simulink library "ammclib_bam_S32K3xx"  (R2016a)
settings: Solver=VariableStepAuto  SolverMode=SingleTasking  StartTime=0.0  StopTime=10.0  RelTol=1e-3
undefined symbols (not defined in the file or in its folder): a1, a2, ADCMaxError, autoCalcEn, b0, b1, b2, cfg, dgain, escale, f16A1, f16A2, f16ADCMaxError, f16B0, f16B1, f16B2, f16C1, f16CC1sc, f16CC1sc_D, f16CC1sc_Q, f16CC2sc, f16CC2sc_D, f16CC2sc_Q, f16DerivGain, f16EGain, f16FiltCoef, f16HystOff, f16HystOn, f16IGain, f16IntegGain, f16IntegGain_D, f16IntegGain_Q, f16IntegGainQ, f16Kd, f16KLs, f16Kq, f16KRs, f16Limit, f16LowerLimit, f16LowerLimit_D, f16LowerLimit_Q, f16LowerLimitQ, f16ModIndex, f16OutValOff, f16OutValOn, f16PropGain, f16PropGain_D, f16PropGain_Q, f16PropGainQ, f16RampDown, f16RampUp, f16UGain, f16UpperLimit, f16UpperLimit_D, f16UpperLimit_Q, f16UpperLimitQ, f16WIGain, f32A1, f32A2, f32ADCMaxError ... (+180)
(part 2 of 50)

== system ammclib_bam_S32K3xx/AMCLIB/F16 ==
  AMCLIB_BemfObsrvDQ_F16 : Subsystem  StartFcn=|  TreatAsAtomicUnit=on  mask(AMCLIB_BemfObsrvDQ_F16){showStates=Hide (faster execution), resetStatesEnable=Pre-set according to the first set of inputs after reset, SampleTime=-1, intmethod=Trapezoidal, if0=350, iksi=1, Ld=3e-4, Lq=3e-4, Rs=0.33, mechspeed=3000, polepairs=1, uscale=15, escale=15, iscale=10, autoCalcEn=on, f16IGain=0, f16UGain=0, f16WIGain=0, f16EGain=0, s16Shift=0, f16CC1sc_D=0, f16CC2sc_D=0, f16UpperLimit_D=0, f16LowerLimit_D=0, f16CC1sc_Q=0, f16CC2sc_Q=0, f16UpperLimit_Q=0, f16LowerLimit_Q=0, u16NShift=0, SampleTime_1=NaN}
      | ts=get_param(gcb,'CompiledSampleTime');
      | if iscell(ts)
      |   ts=ts{1};
      |   if iscell(ts)
      |     ts=ts{1};
      |   end
      | end
      | ts=ts(1);
      | set_param(gcb,'SampleTime_1',num2str(ts));
      | p=Simulink.Mask.get(gcb);
      | hintText=p.getDialogControl('timeHint');
      | SampleTime=Simulink.data.evalinGlobal(bdroot,get_param(gcb,'SampleTime'));
      | p=Simulink.Mask.get(gcb);
      | autoCalcEn=get_param(gcb,'autoCalcEn');
      | if strcmp(autoCalcEn,'on')
      |   if SampleTime==-1
      |     hintText.Prompt='Caution: Implementation parameters depend on inherited sample time. Make sure that the sample time of the block''s inputs corresponds to the sampling period in the target application.';
      |   else
      |     hintText.Prompt='Caution: Implementation parameters depend on the sample time. Make sure that the simulation time step corresponds to the sampling period in the target application.';
      |   end
      |   SampleTime=ts;
      |   f16IGain_bkup=get_param(gcb,'f16IGain');
      |   f16UGain_bkup=get_param(gcb,'f16UGain');
      |   f16WIGain_bkup=get_param(gcb,'f16WIGain');
      |   f16EGain_bkup=get_param(gcb,'f16EGain');
      |   s16Shift_bkup=get_param(gcb,'s16Shift');
      |   f16CC1sc_D_bkup=get_param(gcb,'f16CC1sc_D');
      |   f16CC2sc_D_bkup=get_param(gcb,'f16CC2sc_D');
      |   f16UpperLimit_D_bkup=get_param(gcb,'f16UpperLimit_D');
      |   f16LowerLimit_D_bkup=get_param(gcb,'f16LowerLimit_D');
      |   f16CC1sc_Q_bkup=get_param(gcb,'f16CC1sc_Q');
      |   f16CC2sc_Q_bkup=get_param(gcb,'f16CC2sc_Q');
      |   f16UpperLimit_Q_bkup=get_param(gcb,'f16UpperLimit_Q');
      |   f16LowerLimit_Q_bkup=get_param(gcb,'f16LowerLimit_Q');
      |   u16NShift_bkup=get_param(gcb,'u16NShift');
      |   intmethod=get_param(gcb,'intmethod');
      |   if0=Simulink.data.evalinGlobal(bdroot,get_param(gcb,'if0'));
      |   iksi=Simulink.data.evalinGlobal(bdroot,get_param(gcb,'iksi'));
      |   Ld=Simulink.data.evalinGlobal(bdroot,get_param(gcb,'Ld'));
      |   Lq=Simulink.data.evalinGlobal(bdroot,get_param(gcb,'Lq'));
      |   Rs=Simulink.data.evalinGlobal(bdroot,get_param(gcb,'Rs'));
      |   mechspeed=Simulink.data.evalinGlobal(bdroot,get_param(gcb,'mechspeed'));
      |   polepairs=Simulink.data.evalinGlobal(bdroot,get_param(gcb,'polepairs'));
      |   uscale=Simulink.data.evalinGlobal(bdroot,get_param(gcb,'uscale'));
      |   escale=Simulink.data.evalinGlobal(bdroot,get_param(gcb,'escale'));
      |   iscale=Simulink.data.evalinGlobal(bdroot,get_param(gcb,'iscale'));
      |   if (if0<=0)
      |     warning('Natural frequency f0 must be positive.');
      |   end
      |   if (iksi<=0)
      |     warning('Current loop attenuation must be positive.');
      |   end
      |   if (iksi>1)
      |     warning('Current loop attenuation must not exceed 1.');
      |   end
      |   if (Ld<=0)
      |     warning('Inductance Ld must be positive.');
      |   end
      |   if (Lq<=0)
      |     warning('Inductance Lq must be positive.');
      |   end
      |   if (Rs<0)
      |     warning('Resistance Rs must be non-negative.');
      |   end
      |   if (mechspeed<=0)
      |     warning('Max. speed must be positive.');
      |   end
      |   if (polepairs<1)
      |     warning('Number of pole pairs must be a natural number (1, 2, 3, ...).');
      |   end
      |   if (round(polepairs)~=polepairs)
      |     warning('Number of pole pairs must be a natural number (1, 2, 3, ...).');
      |   end
      |   if (uscale<=0)
      |     warning('U_max must be positive.');
      |   end
      |   if (uscale>escale)
      |     warning('U_max must not exceed E_max');
      |   end
      |   if (iscale<=0)
      |     warning('I_max must be positive.');
      |   end
      |   if (escale<=0)
      |     warning('E_max must be positive.');
      |   end
      |   w0=6.283185307179586*if0;
      |   pgain=2.0*iksi*w0*Ld-Rs;
      |   igain=w0*w0*Ld;
      |   if strcmp(intmethod,'Forward Rectangular')
      |     cc1=pgain;
      |     cc2=-pgain+igain*SampleTime;
      |   else
      |     if strcmp(intmethod,'Backward Rectangular')
      |       cc1=pgain+igain*SampleTime;
      |       cc2=-pgain;
      |     else
      |       cc1=pgain+igain*SampleTime*0.5;
      |       cc2=-pgain+igain*SampleTime*0.5;
      |     end
      |   end
      |   cc1f=cc1*iscale/escale;
      |   cc2f=cc2*iscale/escale;
      |   u16NShift=ceil(log2(abs(cc1f)));
      |   tmpsh=ceil(log2(abs(cc2f)));
      |   if u16NShift<tmpsh
      |     u16NShift=tmpsh;
      |   end
      |   if u16NShift<0
      |     u16NShift=0;
      |   end
      |   if u16NShift>15
      |     u16NShift=15;
      |     warning(['Parameter u16NShift of ' gcb ' exceeds the fixed-point range.']);
      |   end
      |   f16CC1sc_D=round(cc1f*2^(-u16NShift)*2^15);
      |   if f16CC1sc_D>2^15-1
      |     f16CC1sc_D=2^15-1;
      |     warning(['Parameter f16CC1sc_D of ' gcb ' exceeds the fixed-point range.']);
      |   end
      |   if f16CC1sc_D<-2^15
      |     f16CC1sc_D=-2^15;
      |     warning(['Parameter f16CC1sc_D of ' gcb ' exceeds the fixed-point range.']);
      |   end
      |   f16CC2sc_D=round(cc2f*2^(-u16NShift)*2^15);
      |   if f16CC2sc_D>2^15-1
      |     f16CC2sc_D=2^15-1;
      |     warning(['Parameter f16CC2sc_D of ' gcb ' exceeds the fixed-point range.']);
      |   end
      |   if f16CC2sc_D<-2^15
      |     f16CC2sc_D=-2^15;
      |     warning(['Parameter f16CC2sc_D of ' gcb ' exceeds the fixed-point range.']);
      |   end
      |   f16LowerLimit_D=-32768;
      |   f16UpperLimit_D=32767;
      |   f16CC1sc_Q=f16CC1sc_D;
      |   f16CC2sc_Q=f16CC2sc_D;
      |   f16LowerLimit_Q=f16LowerLimit_D;
      |   f16UpperLimit_Q=f16UpperLimit_D;
      |   wmax=polepairs*mechspeed*1.047197551196598e-01;
      |   igainsc=(2.0*Ld-SampleTime*Rs)/(2.0*Ld+SampleTime*Rs);
      |   ugainsc=SampleTime/(2.0*Ld+SampleTime*Rs)*uscale/iscale;
      |   wigainsc=SampleTime*Lq/(2.0*Ld+SampleTime*Rs)*wmax;
      |   egainsc=SampleTime/(2.0*Ld+SampleTime*Rs)*escale/iscale;
      |   maxgain=max(abs([ugainsc,wigainsc,egainsc]));
      |   s16Shift=ceil(log2(abs(maxgain)));
      |   if s16Shift<-15
      |     s16Shift=-15;
      |   end
      |   if s16Shift>15
      |     s16Shift=15;
      |     warning(['Parameter s16Shift of ' gcb ' exceeds the fixed-point range.']);
      |   end
      |   f16IGain=round(igainsc*2^15);
      |   if f16IGain>2^15-1
      |     f16IGain=2^15-1;
      |     warning(['Parameter f16IGain of ' gcb ' exceeds the fixed-point range.']);
      |   end
      |   if f16IGain<-2^15
      |     f16IGain=-2^15;
      |     warning(['Parameter f16IGain of ' gcb ' exceeds the fixed-point range.']);
      |   end
      |   f16UGain=round(ugainsc*2^(-s16Shift)*2^15);
      |   if f16UGain>2^15-1
      |     f16UGain=2^15-1;
      |     warning(['Parameter f16UGain of ' gcb ' exceeds the fixed-point range.']);
      |   end
      |   if f16UGain<-2^15
      |     f16UGain=-2^15;
      |     warning(['Parameter f16UGain of ' gcb ' exceeds the fixed-point range.']);
      |   end
      |   f16WIGain=round(wigainsc*2^(-s16Shift)*2^15);
      |   if f16WIGain>2^15-1
      |     f16WIGain=2^15-1;
      |     warning(['Parameter f16WIGain of ' gcb ' exceeds the fixed-point range.']);
      |   end
      |   if f16WIGain<-2^15
      |     f16WIGain=-2^15;
      |     warning(['Parameter f16WIGain of ' gcb ' exceeds the fixed-point range.']);
      |   end
      |   f16EGain=round(egainsc*2^(-s16Shift)*2^15);
      |   if f16EGain>2^15-1
      |     f16EGain=2^15-1;
      |     warning(['Parameter f16EGain of ' gcb ' exceeds the fixed-point range.']);
      |   end
      |   if f16EGain<-2^15
      |     f16EGain=-2^15;
      |     warning(['Parameter f16EGain of ' gcb ' exceeds the fixed-point range.']);
      |   end
      |   if isnan(f16IGain)
      |     if ~strcmp(f16IGain_bkup,'0')
      |       set_param(gcb,'f16IGain','0');
      |     end
      |   else
      |     tmps=num2str(f16IGain);
      |     if ~strcmp(f16IGain_bkup,tmps)
      |       set_param(gcb,'f16IGain',tmps);
      |     end
      |   end
      |   if isnan(f16UGain)
      |     if ~strcmp(f16UGain_bkup,'0')
      |       set_param(gcb,'f16UGain','0');
      |     end
      |   else
      |     tmps=num2str(f16UGain);
      |     if ~strcmp(f16UGain_bkup,tmps)
      |       set_param(gcb,'f16UGain',tmps);
      |     end
      |   end
      |   if isnan(f16WIGain)
      |     if ~strcmp(f16WIGain_bkup,'0')
      |       set_param(gcb,'f16WIGain','0');
      |     end
      |   else
      |     tmps=num2str(f16WIGain);
      |     if ~strcmp(f16WIGain_bkup,tmps)
      |       set_param(gcb,'f16WIGain',tmps);
      |     end
      |   end
      |   if isnan(f16EGain)
      |     if ~strcmp(f16EGain_bkup,'0')
      |       set_param(gcb,'f16EGain','0');
      |     end
      |   else
      |     tmps=num2str(f16EGain);
      |     if ~strcmp(f16EGain_bkup,tmps)
      |       set_param(gcb,'f16EGain',tmps);
      |     end
      |   end
      |   if isnan(s16Shift)
      |     if ~strcmp(s16Shift_bkup,'0')
      |       set_param(gcb,'s16Shift','0');
      |     end
      |   else
      |     tmps=num2str(s16Shift);
      |     if ~strcmp(s16Shift_bkup,tmps)
      |       set_param(gcb,'s16Shift',tmps);
      |     end
      |   end
      |   if isnan(f16CC1sc_D)
      |     if ~strcmp(f16CC1sc_D_bkup,'0')
      |       set_param(gcb,'f16CC1sc_D','0');
      |     end
      |   else
      |     tmps=num2str(f16CC1sc_D);
      |     if ~strcmp(f16CC1sc_D_bkup,tmps)
      |       set_param(gcb,'f16CC1sc_D',tmps);
      |     end
      |   end
      |   if isnan(f16CC2sc_D)
      |     if ~strcmp(f16CC2sc_D_bkup,'0')
      |       set_param(gcb,'f16CC2sc_D','0');
      |     end
      |   else
      |     tmps=num2str(f16CC2sc_D);
      |     if ~strcmp(f16CC2sc_D_bkup,tmps)
      |       set_param(gcb,'f16CC2sc_D',tmps);
      |     end
      |   end
      |   if isnan(f16UpperLimit_D)
      |     if ~strcmp(f16UpperLimit_D_bkup,'0')
      |       set_param(gcb,'f16UpperLimit_D','0');
      |     end
      |   else
      |     tmps=num2str(f16UpperLimit_D);
      |     if ~strcmp(f16UpperLimit_D_bkup,tmps)
      |       set_param(gcb,'f16UpperLimit_D',tmps);
      |     end
      |   end
      |   if isnan(f16LowerLimit_D)
      |     if ~strcmp(f16LowerLimit_D_bkup,'0')
      |       set_param(gcb,'f16LowerLimit_D','0');
      |     end
      |   else
      |     tmps=num2str(f16LowerLimit_D);
      |     if ~strcmp(f16LowerLimit_D_bkup,tmps)
      |       set_param(gcb,'f16LowerLimit_D',tmps);
      |     end
      |   end
      |   if isnan(f16CC1sc_Q)
      |     if ~strcmp(f16CC1sc_Q_bkup,'0')
      |       set_param(gcb,'f16CC1sc_Q','0');
      |     end
      |   else
      |     tmps=num2str(f16CC1sc_Q);
      |     if ~strcmp(f16CC1sc_Q_bkup,tmps)
      |       set_param(gcb,'f16CC1sc_Q',tmps);
      |     end
      |   end
      |   if isnan(f16CC2sc_Q)
      |     if ~strcmp(f16CC2sc_Q_bkup,'0')
      |       set_param(gcb,'f16CC2sc_Q','0');
      |     end
      |   else
      |     tmps=num2str(f16CC2sc_Q);
      |     if ~strcmp(f16CC2sc_Q_bkup,tmps)
      |       set_param(gcb,'f16CC2sc_Q',tmps);
      |     end
      |   end
      |   if isnan(f16UpperLimit_Q)
      |     if ~strcmp(f16UpperLimit_Q_bkup,'0')
      |       set_param(gcb,'f16UpperLimit_Q','0');
      |     end
      |   else
      |     tmps=num2str(f16UpperLimit_Q);
      |     if ~strcmp(f16UpperLimit_Q_bkup,tmps)
      |       set_param(gcb,'f16UpperLimit_Q',tmps);
      |     end
      |   end
      |   if isnan(f16LowerLimit_Q)
      |     if ~strcmp(f16LowerLimit_Q_bkup,'0')
      |       set_param(gcb,'f16LowerLimit_Q','0');
      |     end
      |   else
      |     tmps=num2str(f16LowerLimit_Q);
      |     if ~strcmp(f16LowerLimit_Q_bkup,tmps)
      |       set_param(gcb,'f16LowerLimit_Q',tmps);
      |     end
      |   end
      |   if isnan(u16NShift)
      |     if ~strcmp(u16NShift_bkup,'0')
      |       set_param(gcb,'u16NShift','0');
      |     end
      |   else
      |     tmps=num2str(u16NShift);
      |     if ~strcmp(u16NShift_bkup,tmps)
      |       set_param(gcb,'u16NShift',tmps);
      |     end
      |   end
      | end
      mask prompts: showStates "Show internal states:"; resetStatesEnable "Internal state after reset:"; SampleTime "Sample time (-1 for inherited):"; intmethod "Integration method:"; if0 "Current loop natural frequency f0 [Hz]:"; iksi "Current loop attenuation ξ:"; Ld "D-axis stator inductance Ld [H]"; Lq "Q-axis stator inductance Lq [H]"; Rs "Winding resistance Rs [ohm]:"; mechspeed "Maximum mechanical speed of the motor [RPM]:"; polepairs "Number of pole pairs of the motor:"; uscale "U_max (maximum DC bus voltage) [V]:"; escale "E_max (maximum back-EMF voltage, same as DC bus if not using field weakening) [V]:"; iscale "I_max (maximum phase current) [A]:"; autoCalcEn "Calculate implementation parameters from physical parameters"; f16IGain "f16IGain (Scaled RL circuit constant):"; f16UGain "f16UGain (Scaled voltage cross-coupling constant):"; f16WIGain "f16WIGain (Scaled angular velocity cross-coupling constant):"; f16EGain "f16EGain (Scaled back-EMF cross-coupling constant):"; s16Shift "s16Shift (Scaling bitwise shift applied to all cross-coupling constants):"; f16CC1sc_D "f16CC1sc_D (CC1 coefficient of the D-axis PI controller):"; f16CC2sc_D "f16CC2sc_D (CC2 coefficient of the D-axis PI controller):"; f16UpperLimit_D "f16UpperLimit_D (Upper Limit of the D-axis PI controller):"; f16LowerLimit_D "f16LowerLimit_D (Lower Limit of the D-axis PI controller):"; f16CC1sc_Q "f16CC1sc_Q (CC1 coefficient of the Q-axis PI controller):"; f16CC2sc_Q "f16CC2sc_Q (CC2 coefficient of the Q-axis PI controller):"; f16UpperLimit_Q "f16UpperLimit_Q (Upper Limit of the Q-axis PI controller):"; f16LowerLimit_Q "f16LowerLimit_Q (Lower Limit of the Q-axis PI controller):"; u16NShift "u16NShift (Scaling bitwise shift applied to the controller coefficients):"; SampleTime_1 "Discrete sample time:"
      mask help: PMSM back-EMF observer DQ in 16-bit fixed-point fractional implementation. This block supports re-initialization of the internal state during simulation. If the block is reset, the observer will align with the motor's position and speed measured in the next time step. This allows seamless on-the-fly transition to the closed-loop control. Refer to the AMMCLIB User's Guide for further details.
      mask init:
      | ddName = get_param(bdroot,'DataDictionary');
      | if length(ddName)==0
      |   set_param(bdroot,'DataDictionary','ammclib_types.sldd');
      | else
      |   dd = Simulink.data.dictionary.open(ddName);
      |   data = getSection(dd,'Design Data');
      |   if ~exist(data,'SWLIBS_2Syst_F16')
      |     addDataSource(dd,'ammclib_types.sldd');
      |     saveChanges(dd);
      |   end
      | end
      | 
      | if showStates == 1
      |   % hidden state variables
      |   if strcmp(get_param([gcb '/f16IGain'], 'BlockType'), 'Inport')
      |     posblk = get_param(gcb, 'Position');
      | 
      |     pos = get_param([gcb, '/f16IGain'], 'Position');
      |     orient = get_param([gcb, '/f16IGain'], 'Orientation');
      |     delete_block([gcb, '/f16IGain']);
      |     add_block('built-in/Ground', [gcb, '/f16IGain'], 'Position', pos, 'Orientation', orient);
      | 
      |     pos = get_param([gcb, '/f16UGain'], 'Position');
      |     orient = get_param([gcb, '/f16UGain'], 'Orientation');
      |     delete_block([gcb, '/f16UGain']);
      |     add_block('built-in/Ground', [gcb, '/f16UGain'], 'Position', pos, 'Orientation', orient);
      | 
      |     pos = get_param([gcb, '/f16WIGain'], 'Position');
      |     orient = get_param([gcb, '/f16WIGain'], 'Orientation');
      |     delete_block([gcb, '/f16WIGain']);
      |     add_block('built-in/Ground', [gcb, '/f16WIGain'], 'Position', pos, 'Orientation', orient);
      | 
      |     pos = get_param([gcb, '/f16EGain'], 'Position');
      |     orient = get_param([gcb, '/f16EGain'], 'Orientation');
      |     delete_block([gcb, '/f16EGain']);
      |     add_block('built-in/Ground', [gcb, '/f16EGain'], 'Position', pos, 'Orientation', orient);
      | 
      |     pos = get_param([gcb, '/s16Shift'], 'Position');
      |     orient = get_param([gcb, '/s16Shift'], 'Orientation');
      |     delete_block([gcb, '/s16Shift']);
      |     add_block('built-in/Ground', [gcb, '/s16Shift'], 'Position', pos, 'Orientation', orient);
      | 
      |     pos = get_param([gcb, '/f16CC1sc_D'], 'Position');
      |     orient = get_param([gcb, '/f16CC1sc_D'], 'Orientation');
      |     delete_block([gcb, '/f16CC1sc_D']);
      |     add_block('built-in/Ground', [gcb, '/f16CC1sc_D'], 'Position', pos, 'Orientation', orient);
      | 
      |     pos = get_param([gcb, '/f16CC2sc_D'], 'Position');
      |     orient = get_param([gcb, '/f16CC2sc_D'], 'Orientation');
      |     delete_block([gcb, '/f16CC2sc_D']);
      |     add_block('built-in/Ground', [gcb, '/f16CC2sc_D'], 'Position', pos, 'Orientation', orient);
      | 
      |     pos = get_param([gcb, '/f16UpperLimit_D'], 'Position');
      |     orient = get_param([gcb, '/f16UpperLimit_D'], 'Orientation');
      |     delete_block([gcb, '/f16UpperLimit_D']);
      |     add_block('built-in/Ground', [gcb, '/f16UpperLimit_D'], 'Position', pos, 'Orientation', orient);
      | 
      |     pos = get_param([gcb, '/f16LowerLimit_D'], 'Position');
      |     orient = get_param([gcb, '/f16LowerLimit_D'], 'Orientation');
      |     delete_block([gcb, '/f16LowerLimit_D']);
      |     add_block('built-in/Ground', [gcb, '/f16LowerLimit_D'], 'Position', pos, 'Orientation', orient);
      | 
      |     pos = get_param([gcb, '/f16CC1sc_Q'], 'Position');
      |     orient = get_param([gcb, '/f16CC1sc_Q'], 'Orientation');
      |     delete_block([gcb, '/f16CC1sc_Q']);
      |     add_block('built-in/Ground', [gcb, '/f16CC1sc_Q'], 'Position', pos, 'Orientation', orient);
      | 
      |     pos = get_param([gcb, '/f16CC2sc_Q'], 'Position');
      |     orient = get_param([gcb, '/f16CC2sc_Q'], 'Orientation');
      |     delete_block([gcb, '/f16CC2sc_Q']);
      |     add_block('built-in/Ground', [gcb, '/f16CC2sc_Q'], 'Position', pos, 'Orientation', orient);
      | 
      |     pos = get_param([gcb, '/f16UpperLimit_Q'], 'Position');
      |     orient = get_param([gcb, '/f16UpperLimit_Q'], 'Orientation');
      |     delete_block([gcb, '/f16UpperLimit_Q']);
      |     add_block('built-in/Ground', [gcb, '/f16UpperLimit_Q'], 'Position', pos, 'Orientation', orient);
      | 
      |     pos = get_param([gcb, '/f16LowerLimit_Q'], 'Position');
      |     orient = get_param([gcb, '/f16LowerLimit_Q'], 'Orientation');
      |     delete_block([gcb, '/f16LowerLimit_Q']);
      |     add_block('built-in/Ground', [gcb, '/f16LowerLimit_Q'], 'Position', pos, 'Orientation', orient);
      | 
      |     pos = get_param([gcb, '/u16NShift'], 'Position');
      |     orient = get_param([gcb, '/u16NShift'], 'Orientation');
      |     delete_block([gcb, '/u16NShift']);
      |     add_block('built-in/Ground', [gcb, '/u16NShift'], 'Position', pos, 'Orientation', orient);
      | 
      |     pos = get_param([gcb, '/f32Acc_D'], 'Position');
      |     orient = get_param([gcb, '/f32Acc_D'], 'Orientation');
      |     delete_block([gcb, '/f32Acc_D']);
      |     add_block('built-in/Ground', [gcb, '/f32Acc_D'], 'Position', pos, 'Orientation', orient);
      | 
      |     pos = get_param([gcb, '/f16InErrK1_D'], 'Position');
      |     orient = get_param([gcb, '/f16InErrK1_D'], 'Orientation');
      |     delete_block([gcb, '/f16InErrK1_D']);
      |     add_block('built-in/Ground', [gcb, '/f16InErrK1_D'], 'Position', pos, 'Orientation', orient);
      | 
      |     pos = get_param([gcb, '/f32Acc_Q'], 'Position');
      |     orient = get_param([gcb, '/f32Acc_Q'], 'Orientation');
      |     delete_block([gcb, '/f32Acc_Q']);
      |     add_block('built-in/Ground', [gcb, '/f32Acc_Q'], 'Position', pos, 'Orientation', orient);
      | 
      |     pos = get_param([gcb, '/f16InErrK1_Q'], 'Position');
      |     orient = get_param([gcb, '/f16InErrK1_Q'], 'Orientation');
      |     delete_block([gcb, '/f16InErrK1_Q']);
      |     add_block('built-in/Ground', [gcb, '/f16InErrK1_Q'], 'Position', pos, 'Orientation', orient);
      | 
      |     pos = get_param([gcb, '/f32IObsrvIn_1L_D'], 'Position');
      |     orient = get_param([gcb, '/f32IObsrvIn_1L_D'], 'Orientation');
      |     delete_block([gcb, '/f32IObsrvIn_1L_D']);
      |     add_block('built-in/Ground', [gcb, '/f32IObsrvIn_1L_D'], 'Position', pos, 'Orientation', orient);
      | 
      |     pos = get_param([gcb, '/f16IObsrvIn_1H_D'], 'Position');
      |     orient = get_param([gcb, '/f16IObsrvIn_1H_D'], 'Orientation');
      |     delete_block([gcb, '/f16IObsrvIn_1H_D']);
      |     add_block('built-in/Ground', [gcb, '/f16IObsrvIn_1H_D'], 'Position', pos, 'Orientation', orient);
      | 
      |     pos = get_param([gcb, '/f32IObsrvIn_1L_Q'], 'Position');
      |     orient = get_param([gcb, '/f32IObsrvIn_1L_Q'], 'Orientation');
      |     delete_block([gcb, '/f32IObsrvIn_1L_Q']);
      |     add_block('built-in/Ground', [gcb, '/f32IObsrvIn_1L_Q'], 'Position', pos, 'Orientation', orient);
      | 
      |     pos = get_param([gcb, '/f16IObsrvIn_1H_Q'], 'Position');
      |     orient = get_param([gcb, '/f16IObsrvIn_1H_Q'], 'Orientation');
      |     delete_block([gcb, '/f16IObsrvIn_1H_Q']);
      |     add_block('built-in/Ground', [gcb, '/f16IObsrvIn_1H_Q'], 'Position', pos, 'Orientation', orient);
      | 
      |     pos = get_param([gcb, '/f32IObsrv_D'], 'Position');
      |     orient = get_param([gcb, '/f32IObsrv_D'], 'Orientation');
      |     delete_block([gcb, '/f32IObsrv_D']);
      |     add_block('built-in/Ground', [gcb, '/f32IObsrv_D'], 'Position', pos, 'Orientation', orient);
      | 
      |     pos = get_param([gcb, '/f32IObsrv_Q'], 'Position');
      |     orient = get_param([gcb, '/f32IObsrv_Q'], 'Orientation');
      |     delete_block([gcb, '/f32IObsrv_Q']);
      |     add_block('built-in/Ground', [gcb, '/f32IObsrv_Q'], 'Position', pos, 'Orientation', orient);
      | 
      | 
      |     pmask=Simulink.Mask.get(gcb);
      |     pctrl=pmask.getParameter('SampleTime');
      |     pctrl.set('TypeOptions',{'pIAB/SampleTime','pUAB/SampleTime','f16Velocity/SampleTime','f16Phase/SampleTime'});
      | 
      |     pos = get_param([gcb '/f16EObsrv_D_Out'], 'Position');
      |     orient = get_param([gcb '/f16EObsrv_D_Out'], 'Orientation');
      |     delete_block([gcb '/f16EObsrv_D_Out']);
      |     add_block('built-in/Terminator', [gcb '/f16EObsrv_D_Out'], 'Position', pos, 'Orientation', orient);
      | 
      |     pos = get_param([gcb '/f16EObsrv_Q_Out'], 'Position');
      |     orient = get_param([gcb '/f16EObsrv_Q_Out'], 'Orientation');
      |     delete_block([gcb '/f16EObsrv_Q_Out']);
      |     add_block('built-in/Terminator', [gcb '/f16EObsrv_Q_Out'], 'Position', pos, 'Orientation', orient);
      | 
      |     pos = get_param([gcb '/f32Acc_D_Out'], 'Position');
      |     orient = get_param([gcb '/f32Acc_D_Out'], 'Orientation');
      |     delete_block([gcb '/f32Acc_D_Out']);
      |     add_block('built-in/Terminator', [gcb '/f32Acc_D_Out'], 'Position', pos, 'Orientation', orient);
      | 
      |     pos = get_param([gcb '/f16InErrK1_D_Out'], 'Position');
      |     orient = get_param([gcb '/f16InErrK1_D_Out'], 'Orientation');
      |     delete_block([gcb '/f16InErrK1_D_Out']);
      |     add_block('built-in/Terminator', [gcb '/f16InErrK1_D_Out'], 'Position', pos, 'Orientation', orient);
      | 
      |     pos = get_param([gcb '/f32Acc_Q_Out'], 'Position');
      |     orient = get_param([gcb '/f32Acc_Q_Out'], 'Orientation');
      |     delete_block([gcb '/f32Acc_Q_Out']);
      |     add_block('built-in/Terminator', [gcb '/f32Acc_Q_Out'], 'Position', pos, 'Orientation', orient);
      | 
      |     pos = get_param([gcb '/f16InErrK1_Q_Out'], 'Position');
      |     orient = get_param([gcb '/f16InErrK1_Q_Out'], 'Orientation');
      |     delete_block([gcb '/f16InErrK1_Q_Out']);
      |     add_block('built-in/Terminator', [gcb '/f16InErrK1_Q_Out'], 'Position', pos, 'Orientation', orient);
      | 
      |     pos = get_param([gcb '/f32IObsrvIn_1L_D_Out'], 'Position');
      |     orient = get_param([gcb '/f32IObsrvIn_1L_D_Out'], 'Orientation');
      |     delete_block([gcb '/f32IObsrvIn_1L_D_Out']);
      |     add_block('built-in/Terminator', [gcb '/f32IObsrvIn_1L_D_Out'], 'Position', pos, 'Orientation', orient);
      | 
      |     pos = get_param([gcb '/f16IObsrvIn_1H_D_Out'], 'Position');
      |     orient = get_param([gcb '/f16IObsrvIn_1H_D_Out'], 'Orientation');
      |     delete_block([gcb '/f16IObsrvIn_1H_D_Out']);
      |     add_block('built-in/Terminator', [gcb '/f16IObsrvIn_1H_D_Out'], 'Position', pos, 'Orientation', orient);
      | 
      |     pos = get_param([gcb '/f32IObsrvIn_1L_Q_Out'], 'Position');
      |     orient = get_param([gcb '/f32IObsrvIn_1L_Q_Out'], 'Orientation');
      |     delete_block([gcb '/f32IObsrvIn_1L_Q_Out']);
      |     add_block('built-in/Terminator', [gcb '/f32IObsrvIn_1L_Q_Out'], 'Position', pos, 'Orientation', orient);
      | 
      |     pos = get_param([gcb '/f16IObsrvIn_1H_Q_Out'], 'Position');
      |     orient = get_param([gcb '/f16IObsrvIn_1H_Q_Out'], 'Orientation');
      |     delete_block([gcb '/f16IObsrvIn_1H_Q_Out']);
      |     add_block('built-in/Terminator', [gcb '/f16IObsrvIn_1H_Q_Out'], 'Position', pos, 'Orientation', orient);
      | 
      |     pos = get_param([gcb '/f32IObsrv_D_Out'], 'Position');
      |     orient = get_param([gcb '/f32IObsrv_D_Out'], 'Orientation');
      |     delete_block([gcb '/f32IObsrv_D_Out']);
      |     add_block('built-in/Terminator', [gcb '/f32IObsrv_D_Out'], 'Position', pos, 'Orientation', orient);
      | 
      |     pos = get_param([gcb '/f32IObsrv_Q_Out'], 'Position');
      |     orient = get_param([gcb '/f32IObsrv_Q_Out'], 'Orientation');
      |     delete_block([gcb '/f32IObsrv_Q_Out']);
      |     add_block('built-in/Terminator', [gcb '/f32IObsrv_Q_Out'], 'Position', pos, 'Orientation', orient);
      | 
      |     set_param([gcb '/pIAB'], 'Port', '1');
      |     set_param([gcb '/pUAB'], 'Port', '2');
      |     set_param([gcb '/f16Velocity'], 'Port', '3');
      |     set_param([gcb '/f16Phase'], 'Port', '4');
      | 
      |     tmpOutCnt=0;
      |     tmpOutCnt=tmpOutCnt+1;
      |     set_param([gcb '/f16PhaseErr'], 'Port', num2str(tmpOutCnt));
      | 
      |     autoCalcEn=get_param(gcb,'autoCalcEn');
      |     if strcmp(autoCalcEn,'on')
      |       set_param(gcb,'MaskEnables',{'on','on','on','on','on','on','on','on','on','on','on','on','on','on','on','on','on','on','on','on','on','on','on','on','on','on','on','on','on','off'});
      |     else
      |       set_param(gcb,'MaskEnables',{'on','on','on','off','off','off','off','off','off','off','off','off','off','off','on','on','on','on','on','on','on','on','on','on','on','on','on','on','on','off'});
      |     end
      | 
      |     if (posblk(4) - posblk(2)) > 125
      |       height = 125;
      |       set_param(gcb,'Position',[posblk(1), posblk(2), posblk(3), posblk(2)+height])
      |     end
      |   end
      | else
      |   % shown state variables
      |   if strcmp(get_param([gcb '/f16IGain'], 'BlockType'), 'Ground')
      |     posblk = get_param(gcb, 'Position');
      | 
      |     pos = get_param([gcb, '/f16IGain'], 'Position');
      |     orient = get_param([gcb, '/f16IGain'], 'Orientation');
      |     delete_block([gcb, '/f16IGain']);
      |     add_block('built-in/Inport', [gcb, '/f16IGain'], 'Position', pos, 'Orientation', orient, 'OutDataTypeStr', 'int16');
      | 
      |     pos = get_param([gcb, '/f16UGain'], 'Position');
      |     orient = get_param([gcb, '/f16UGain'], 'Orientation');
      |     delete_block([gcb, '/f16UGain']);
      |     add_block('built-in/Inport', [gcb, '/f16UGain'], 'Position', pos, 'Orientation', orient, 'OutDataTypeStr', 'int16');
      | 
      |     pos = get_param([gcb, '/f16WIGain'], 'Position');
      |     orient = get_param([gcb, '/f16WIGain'], 'Orientation');
      |     delete_block([gcb, '/f16WIGain']);
      |     add_block('built-in/Inport', [gcb, '/f16WIGain'], 'Position', pos, 'Orientation', orient, 'OutDataTypeStr', 'int16');
      | 
      |     pos = get_param([gcb, '/f16EGain'], 'Position');
      |     orient = get_param([gcb, '/f16EGain'], 'Orientation');
      |     delete_block([gcb, '/f16EGain']);
      |     add_block('built-in/Inport', [gcb, '/f16EGain'], 'Position', pos, 'Orientation', orient, 'OutDataTypeStr', 'int16');
      | 
      |     pos = get_param([gcb, '/s16Shift'], 'Position');
      |     orient = get_param([gcb, '/s16Shift'], 'Orientation');
      |     delete_block([gcb, '/s16Shift']);
      |     add_block('built-in/Inport', [gcb, '/s16Shift'], 'Position', pos, 'Orientation', orient, 'OutDataTypeStr', 'int16');
      | 
      |     pos = get_param([gcb, '/f16CC1sc_D'], 'Position');
      |     orient = get_param([gcb, '/f16CC1sc_D'], 'Orientation');
      |     delete_block([gcb, '/f16CC1sc_D']);
      |     add_block('built-in/Inport', [gcb, '/f16CC1sc_D'], 'Position', pos, 'Orientation', orient, 'OutDataTypeStr', 'int16');
      | 
      |     pos = get_param([gcb, '/f16CC2sc_D'], 'Position');
      |     orient = get_param([gcb, '/f16CC2sc_D'], 'Orientation');
      |     delete_block([gcb, '/f16CC2sc_D']);
      |     add_block('built-in/Inport', [gcb, '/f16CC2sc_D'], 'Position', pos, 'Orientation', orient, 'OutDataTypeStr', 'int16');
      | 
      |     pos = get_param([gcb, '/f16UpperLimit_D'], 'Position');
      |     orient = get_param([gcb, '/f16UpperLimit_D'], 'Orientation');
      |     delete_block([gcb, '/f16UpperLimit_D']);
      |     add_block('built-in/Inport', [gcb, '/f16UpperLimit_D'], 'Position', pos, 'Orientation', orient, 'OutDataTypeStr', 'int16');
      | 
      |     pos = get_param([gcb, '/f16LowerLimit_D'], 'Position');
      |     orient = get_param([gcb, '/f16LowerLimit_D'], 'Orientation');
      |     delete_block([gcb, '/f16LowerLimit_D']);
      |     add_block('built-in/Inport', [gcb, '/f16LowerLimit_D'], 'Position', pos, 'Orientation', orient, 'OutDataTypeStr', 'int16');
      | 
      |     pos = get_param([gcb, '/f16CC1sc_Q'], 'Position');
      |     orient = get_param([gcb, '/f16CC1sc_Q'], 'Orientation');
      |     delete_block([gcb, '/f16CC1sc_Q']);
      |     add_block('built-in/Inport', [gcb, '/f16CC1sc_Q'], 'Position', pos, 'Orientation', orient, 'OutDataTypeStr', 'int16');
      | 
      |     pos = get_param([gcb, '/f16CC2sc_Q'], 'Position');
      |     orient = get_param([gcb, '/f16CC2sc_Q'], 'Orientation');
      |     delete_block([gcb, '/f16CC2sc_Q']);
      |     add_block('built-in/Inport', [gcb, '/f16CC2sc_Q'], 'Position', pos, 'Orientation', orient, 'OutDataTypeStr', 'int16');
      | 
      |     pos = get_param([gcb, '/f16UpperLimit_Q'], 'Position');
      |     orient = get_param([gcb, '/f16UpperLimit_Q'], 'Orientation');
      |     delete_block([gcb, '/f16UpperLimit_Q']);
      |     add_block('built-in/Inport', [gcb, '/f16UpperLimit_Q'], 'Position', pos, 'Orientation', orient, 'OutDataTypeStr', 'int16');
      | 
      |     pos = get_param([gcb, '/f16LowerLimit_Q'], 'Position');
      |     orient = get_param([gcb, '/f16LowerLimit_Q'], 'Orientation');
      |     delete_block([gcb, '/f16LowerLimit_Q']);
      |     add_block('built-in/Inport', [gcb, '/f16LowerLimit_Q'], 'Position', pos, 'Orientation', orient, 'OutDataTypeStr', 'int16');
      | 
      |     pos = get_param([gcb, '/u16NShift'], 'Position');
      |     orient = get_param([gcb, '/u16NShift'], 'Orientation');
      |     delete_block([gcb, '/u16NShift']);
      |     add_block('built-in/Inport', [gcb, '/u16NShift'], 'Position', pos, 'Orientation', orient, 'OutDataTypeStr', 'uint16');
      | 
      |     pos = get_param([gcb, '/f32Acc_D'], 'Position');
      |     orient = get_param([gcb, '/f32Acc_D'], 'Orientation');
      |     delete_block([gcb, '/f32Acc_D']);
      |     add_block('built-in/Inport', [gcb, '/f32Acc_D'], 'Position', pos, 'Orientation', orient, 'OutDataTypeStr', 'int32');
      | 
      |     pos = get_param([gcb, '/f16InErrK1_D'], 'Position');
      |     orient = get_param([gcb, '/f16InErrK1_D'], 'Orientation');
      |     delete_block([gcb, '/f16InErrK1_D']);
      |     add_block('built-in/Inport', [gcb, '/f16InErrK1_D'], 'Position', pos, 'Orientation', orient, 'OutDataTypeStr', 'int16');
      | 
      |     pos = get_param([gcb, '/f32Acc_Q'], 'Position');
      |     orient = get_param([gcb, '/f32Acc_Q'], 'Orientation');
      |     delete_block([gcb, '/f32Acc_Q']);
      |     add_block('built-in/Inport', [gcb, '/f32Acc_Q'], 'Position', pos, 'Orientation', orient, 'OutDataTypeStr', 'int32');
      | 
      |     pos = get_param([gcb, '/f16InErrK1_Q'], 'Position');
      |     orient = get_param([gcb, '/f16InErrK1_Q'], 'Orientation');
      |     delete_block([gcb, '/f16InErrK1_Q']);
      |     add_block('built-in/Inport', [gcb, '/f16InErrK1_Q'], 'Position', pos, 'Orientation', orient, 'OutDataTypeStr', 'int16');
      | 
      |     pos = get_param([gcb, '/f32IObsrvIn_1L_D'], 'Position');
      |     orient = get_param([gcb, '/f32IObsrvIn_1L_D'], 'Orientation');
      |     delete_block([gcb, '/f32IObsrvIn_1L_D']);
      |     add_block('built-in/Inport', [gcb, '/f32IObsrvIn_1L_D'], 'Position', pos, 'Orientation', orient, 'OutDataTypeStr', 'int32');
      | 
      |     pos = get_param([gcb, '/f16IObsrvIn_1H_D'], 'Position');
      |     orient = get_param([gcb, '/f16IObsrvIn_1H_D'], 'Orientation');
      |     delete_block([gcb, '/f16IObsrvIn_1H_D']);
      |     add_block('built-in/Inport', [gcb, '/f16IObsrvIn_1H_D'], 'Position', pos, 'Orientation', orient, 'OutDataTypeStr', 'int16');
      | 
      |     pos = get_param([gcb, '/f32IObsrvIn_1L_Q'], 'Position');
      |     orient = get_param([gcb, '/f32IObsrvIn_1L_Q'], 'Orientation');
      |     delete_block([gcb, '/f32IObsrvIn_1L_Q']);
      |     add_block('built-in/Inport', [gcb, '/f32IObsrvIn_1L_Q'], 'Position', pos, 'Orientation', orient, 'OutDataTypeStr', 'int32');
      | 
      |     pos = get_param([gcb, '/f16IObsrvIn_1H_Q'], 'Position');
      |     orient = get_param([gcb, '/f16IObsrvIn_1H_Q'], 'Orientation');
      |     delete_block([gcb, '/f16IObsrvIn_1H_Q']);
      |     add_block('built-in/Inport', [gcb, '/f16IObsrvIn_1H_Q'], 'Position', pos, 'Orientation', orient, 'OutDataTypeStr', 'int16');
      | 
      |     pos = get_param([gcb, '/f32IObsrv_D'], 'Position');
      |     orient = get_param([gcb, '/f32IObsrv_D'], 'Orientation');
      |     delete_block([gcb, '/f32IObsrv_D']);
      |     add_block('built-in/Inport', [gcb, '/f32IObsrv_D'], 'Position', pos, 'Orientation', orient, 'OutDataTypeStr', 'int32');
      | 
      |     pos = get_param([gcb, '/f32IObsrv_Q'], 'Position');
      |     orient = get_param([gcb, '/f32IObsrv_Q'], 'Orientation');
      |     delete_block([gcb, '/f32IObsrv_Q']);
      |     add_block('built-in/Inport', [gcb, '/f32IObsrv_Q'], 'Position', pos, 'Orientation', orient, 'OutDataTypeStr', 'int32');
      | 
      | 
      | 
      |     pos = get_param([gcb '/f16EObsrv_D_Out'], 'Position');
      |     orient = get_param([gcb '/f16EObsrv_D_Out'], 'Orientation');
      |     delete_block([gcb '/f16EObsrv_D_Out']);
      |     add_block('built-in/Outport', [gcb '/f16EObsrv_D_Out'], 'Position', pos, 'Orientation', orient);
      | 
      |     pos = get_param([gcb '/f16EObsrv_Q_Out'], 'Position');
      |     orient = get_param([gcb '/f16EObsrv_Q_Out'], 'Orientation');
      |     delete_block([gcb '/f16EObsrv_Q_Out']);
      |     add_block('built-in/Outport', [gcb '/f16EObsrv_Q_Out'], 'Position', pos, 'Orientation', orient);
      | 
      |     pos = get_param([gcb '/f32Acc_D_Out'], 'Position');
      |     orient = get_param([gcb '/f32Acc_D_Out'], 'Orientation');
      |     delete_block([gcb '/f32Acc_D_Out']);
      |     add_block('built-in/Outport', [gcb '/f32Acc_D_Out'], 'Position', pos, 'Orientation', orient);
      | 
      |     pos = get_param([gcb '/f16InErrK1_D_Out'], 'Position');
      |     orient = get_param([gcb '/f16InErrK1_D_Out'], 'Orientation');
      |     delete_block([gcb '/f16InErrK1_D_Out']);
      |     add_block('built-in/Outport', [gcb '/f16InErrK1_D_Out'], 'Position', pos, 'Orientation', orient);
      | 
      |     pos = get_param([gcb '/f32Acc_Q_Out'], 'Position');
      |     orient = get_param([gcb '/f32Acc_Q_Out'], 'Orientation');
      |     delete_block([gcb '/f32Acc_Q_Out']);
      |     add_block('built-in/Outport', [gcb '/f32Acc_Q_Out'], 'Position', pos, 'Orientation', orient);
      | 
      |     pos = get_param([gcb '/f16InErrK1_Q_Out'], 'Position');
      |     orient = get_param([gcb '/f16InErrK1_Q_Out'], 'Orientation');
      |     delete_block([gcb '/f16InErrK1_Q_Out']);
      |     add_block('built-in/Outport', [gcb '/f16InErrK1_Q_Out'], 'Position', pos, 'Orientation', orient);
      | 
      |     pos = get_param([gcb '/f32IObsrvIn_1L_D_Out'], 'Position');
      |     orient = get_param([gcb '/f32IObsrvIn_1L_D_Out'], 'Orientation');
      |     delete_block([gcb '/f32IObsrvIn_1L_D_Out']);
      |     add_block('built-in/Outport', [gcb '/f32IObsrvIn_1L_D_Out'], 'Position', pos, 'Orientation', orient);
      | 
      |     pos = get_param([gcb '/f16IObsrvIn_1H_D_Out'], 'Position');
      |     orient = get_param([gcb '/f16IObsrvIn_1H_D_Out'], 'Orientation');
      |     delete_block([gcb '/f16IObsrvIn_1H_D_Out']);
      |     add_block('built-in/Outport', [gcb '/f16IObsrvIn_1H_D_Out'], 'Position', pos, 'Orientation', orient);
      | 
      |     pos = get_param([gcb '/f32IObsrvIn_1L_Q_Out'], 'Position');
      |     orient = get_param([gcb '/f32IObsrvIn_1L_Q_Out'], 'Orientation');
      |     delete_block([gcb '/f32IObsrvIn_1L_Q_Out']);
      |     add_block('built-in/Outport', [gcb '/f32IObsrvIn_1L_Q_Out'], 'Position', pos, 'Orientation', orient);
      | 
      |     pos = get_param([gcb '/f16IObsrvIn_1H_Q_Out'], 'Position');
      |     orient = get_param([gcb '/f16IObsrvIn_1H_Q_Out'], 'Orientation');
      |     delete_block([gcb '/f16IObsrvIn_1H_Q_Out']);
      |     add_block('built-in/Outport', [gcb '/f16IObsrvIn_1H_Q_Out'], 'Position', pos, 'Orientation', orient);
      | 
      |     pos = get_param([gcb '/f32IObsrv_D_Out'], 'Position');
      |     orient = get_param([gcb '/f32IObsrv_D_Out'], 'Orientation');
      |     delete_block([gcb '/f32IObsrv_D_Out']);
      |     add_block('built-in/Outport', [gcb '/f32IObsrv_D_Out'], 'Position', pos, 'Orientation', orient);
      | 
      |     pos = get_param([gcb '/f32IObsrv_Q_Out'], 'Position');
      |     orient = get_param([gcb '/f32IObsrv_Q_Out'], 'Orientation');
      |     delete_block([gcb '/f32IObsrv_Q_Out']);
      |     add_block('built-in/Outport', [gcb '/f32IObsrv_Q_Out'], 'Position', pos, 'Orientation', orient);
      | 
      | 
      |     pmask=Simulink.Mask.get(gcb);
      |     pctrl=pmask.getParameter('SampleTime');
      |     pctrl.set('TypeOptions',{'pIAB/SampleTime','pUAB/SampleTime','f16Velocity/SampleTime','f16Phase/SampleTime','f16IGain/SampleTime','f16UGain/SampleTime','f16WIGain/SampleTime','f16EGain/SampleTime','s16Shift/SampleTime','f16CC1sc_D/SampleTime','f16CC2sc_D/SampleTime','f16UpperLimit_D/SampleTime','f16LowerLimit_D/SampleTime','f16CC1sc_Q/SampleTime','f16CC2sc_Q/SampleTime','f16UpperLimit_Q/SampleTime','f16LowerLimit_Q/SampleTime','u16NShift/SampleTime','f32Acc_D/SampleTime','f16InErrK1_D/SampleTime','f32Acc_Q/SampleTime','f16InErrK1_Q/SampleTime','f32IObsrvIn_1L_D/SampleTime','f16IObsrvIn_1H_D/SampleTime','f32IObsrvIn_1L_Q/SampleTime','f16IObsrvIn_1H_Q/SampleTime','f32IObsrv_D/SampleTime','f32IObsrv_Q/SampleTime'});
      | 
      |     set_param([gcb '/pIAB'], 'Port', '1');
      |     set_param([gcb '/pUAB'], 'Port', '2');
      |     set_param([gcb '/f16Velocity'], 'Port', '3');
      |     set_param([gcb '/f16Phase'], 'Port', '4');
      |     set_param([gcb '/f16IGain'], 'Port', '5');
      |     set_param([gcb '/f16UGain'], 'Port', '6');
      |     set_param([gcb '/f16WIGain'], 'Port', '7');
      |     set_param([gcb '/f16EGain'], 'Port', '8');
      |     set_param([gcb '/s16Shift'], 'Port', '9');
      |     set_param([gcb '/f16CC1sc_D'], 'Port', '10');
      |     set_param([gcb '/f16CC2sc_D'], 'Port', '11');
      |     set_param([gcb '/f16UpperLimit_D'], 'Port', '12');
      |     set_param([gcb '/f16LowerLimit_D'], 'Port', '13');
      |     set_param([gcb '/f16CC1sc_Q'], 'Port', '14');
      |     set_param([gcb '/f16CC2sc_Q'], 'Port', '15');
      |     set_param([gcb '/f16UpperLimit_Q'], 'Port', '16');
      |     set_param([gcb '/f16LowerLimit_Q'], 'Port', '17');
      |     set_param([gcb '/u16NShift'], 'Port', '18');
      |     set_param([gcb '/f32Acc_D'], 'Port', '19');
      |     set_param([gcb '/f16InErrK1_D'], 'Port', '20');
      |     set_param([gcb '/f32Acc_Q'], 'Port', '21');
      |     set_param([gcb '/f16InErrK1_Q'], 'Port', '22');
      |     set_param([gcb '/f32IObsrvIn_1L_D'], 'Port', '23');
      |     set_param([gcb '/f16IObsrvIn_1H_D'], 'Port', '24');
      |     set_param([gcb '/f32IObsrvIn_1L_Q'], 'Port', '25');
      |     set_param([gcb '/f16IObsrvIn_1H_Q'], 'Port', '26');
      |     set_param([gcb '/f32IObsrv_D'], 'Port', '27');
      |     set_param([gcb '/f32IObsrv_Q'], 'Port', '28');
      | 
      |     tmpOutCnt=0;
      |     tmpOutCnt=tmpOutCnt+1;
      |     set_param([gcb '/f16PhaseErr'], 'Port', num2str(tmpOutCnt));
      |     tmpOutCnt=tmpOutCnt+1;
      |     set_param([gcb '/f16EObsrv_D_Out'], 'Port', num2str(tmpOutCnt));
      |     tmpOutCnt=tmpOutCnt+1;
      |     set_param([gcb '/f16EObsrv_Q_Out'], 'Port', num2str(tmpOutCnt));
      |     tmpOutCnt=tmpOutCnt+1;
      |     set_param([gcb '/f32Acc_D_Out'], 'Port', num2str(tmpOutCnt));
      |     tmpOutCnt=tmpOutCnt+1;
      |     set_param([gcb '/f16InErrK1_D_Out'], 'Port', num2str(tmpOutCnt));
      |     tmpOutCnt=tmpOutCnt+1;
      |     set_param([gcb '/f32Acc_Q_Out'], 'Port', num2str(tmpOutCnt));
      |     tmpOutCnt=tmpOutCnt+1;
      |     set_param([gcb '/f16InErrK1_Q_Out'], 'Port', num2str(tmpOutCnt));
      |     tmpOutCnt=tmpOutCnt+1;
      |     set_param([gcb '/f32IObsrvIn_1L_D_Out'], 'Port', num2str(tmpOutCnt));
      |     tmpOutCnt=tmpOutCnt+1;
      |     set_param([gcb '/f16IObsrvIn_1H_D_Out'], 'Port', num2str(tmpOutCnt));
      |     tmpOutCnt=tmpOutCnt+1;
      |     set_param([gcb '/f32IObsrvIn_1L_Q_Out'], 'Port', num2str(tmpOutCnt));
      |     tmpOutCnt=tmpOutCnt+1;
      |     set_param([gcb '/f16IObsrvIn_1H_Q_Out'], 'Port', num2str(tmpOutCnt));
      |     tmpOutCnt=tmpOutCnt+1;
      |     set_param([gcb '/f32IObsrv_D_Out'], 'Port', num2str(tmpOutCnt));
      |     tmpOutCnt=tmpOutCnt+1;
      |     set_param([gcb '/f32IObsrv_Q_Out'], 'Port', num2str(tmpOutCnt));
      | 
      |     set_param(gcb,'MaskEnables',{'on','on','on','off','off','off','off','off','off','off','off','off','off','off','off','off','off','off','off','off','off','off','off','off','off','off','off','off','off','off'});
      | 
      |     if (posblk(4) - posblk(2)) < 725
      |       height = 725;
      |       set_param(gcb,'Position',[posblk(1), posblk(2), posblk(3), posblk(2)+height])
      |     end
      |   end
      | end
      settings: RTWSystemCode=Inline
      mask Help: web([fileparts(which('ammclib_bam_S32K3xx.slx')) '/../doc/S32K3XXMCLUG.pdf'], '-browser')
      mask TypeOptions showStates: Hide (faster execution) | Show (allows debugging; connect feedback loops manually)
      mask Callback showStates:
      | maskStr=get_param(gcb,'showStates');
      | if strcmp(maskStr,'Hide (faster execution)')
      |   if strcmp(get_param([gcb '/f16IGain'], 'BlockType'), 'Inport')
      |     autoCalcEn=get_param(gcb,'autoCalcEn');
      |     if strcmp(autoCalcEn,'on')
      |       set_param(gcb,'MaskEnables',{'on','on','on','on','on','on','on','on','on','on','on','on','on','on','on','on','on','on','on','on','on','on','on','on','on','on','on','on','on','off'});
      |     else
      |       set_param(gcb,'MaskEnables',{'on','on','on','off','off','off','off','off','off','off','off','off','off','off','on','on','on','on','on','on','on','on','on','on','on','on','on','on','on','off'});
      |     end
      |   end
      | else
      |   if strcmp(get_param([gcb '/f16IGain'], 'BlockType'), 'Ground')
      |     set_param(gcb,'MaskEnables',{'on','on','on','off','off','off','off','off','off','off','off','off','off','off','off','off','off','off','off','off','off','off','off','off','off','off','off','off','off','off'});
      |   end
      | end
      mask TypeOptions resetStatesEnable: Pre-set according to the first set of inputs after reset | Clear to zero
      mask TypeOptions SampleTime: pIAB/SampleTime | pUAB/SampleTime | f16Velocity/SampleTime | f16Phase/SampleTime
      mask Callback SampleTime:
      | p=Simulink.Mask.get(gcb);
      | hintText=p.getDialogControl('timeHint');
      | SampleTime=Simulink.data.evalinGlobal(bdroot,get_param(gcb,'SampleTime'));
      | SampleTime_1=str2double(get_param(gcb,'SampleTime_1'));
      | if (((SampleTime==-1) && (~contains(hintText.Prompt,'inherited'))) || ...
      |     ((SampleTime~=-1) && contains(hintText.Prompt,'inherited')) || ...
      |     ((SampleTime~=-1) && (SampleTime_1~=SampleTime)) || ...
      |     ((SampleTime_1~=-1) && contains(hintText.Prompt,'yet')))
      |   if ((SampleTime==-1) && (~contains(hintText.Prompt,'inherited')))
      |     set_param(gcb,'SampleTime_1',num2str(NaN));
      |     SampleTime_1=NaN;
      |   end
      |   if (SampleTime~=-1)
      |     set_param(gcb,'SampleTime_1',num2str(SampleTime));
      |     SampleTime_1=SampleTime;
      |   end
      |   autoCalcEn=get_param(gcb,'autoCalcEn');
      |   if strcmp(autoCalcEn,'on')
      |     p=Simulink.Mask.get(gcb);
      |     hintText=p.getDialogControl('timeHint');
      |     if SampleTime==-1
      |       SampleTime=SampleTime_1;
      |       if isnan(SampleTime)
      |         hintText.Prompt='Note: Implementation parameters cannot be calculated yet because the block''s inherited sample time is unknown. Simulink will update the sample time when you run the simulation.';
      |       else
      |         hintText.Prompt='Caution: Implementation parameters depend on inherited sample time. Make sure that the sample time of the block''s inputs corresponds to the sampling period in the target application.';
      |       end
      |     else
      |       hintText.Prompt='Caution: Implementation parameters depend on the sample time. Make sure that the simulation time step corresponds to the sampling period in the target application.';
      |     end
      |     f16IGain_bkup=get_param(gcb,'f16IGain');
      |     f16UGain_bkup=get_param(gcb,'f16UGain');
      |     f16WIGain_bkup=get_param(gcb,'f16WIGain');
      |     f16EGain_bkup=get_param(gcb,'f16EGain');
      |     s16Shift_bkup=get_param(gcb,'s16Shift');
      |     f16CC1sc_D_bkup=get_param(gcb,'f16CC1sc_D');
      |     f16CC2sc_D_bkup=get_param(gcb,'f16CC2sc_D');
      |     f16UpperLimit_D_bkup=get_param(gcb,'f16UpperLimit_D');
      |     f16LowerLimit_D_bkup=get_param(gcb,'f16LowerLimit_D');
      |     f16CC1sc_Q_bkup=get_param(gcb,'f16CC1sc_Q');
      |     f16CC2sc_Q_bkup=get_param(gcb,'f16CC2sc_Q');
      |     f16UpperLimit_Q_bkup=get_param(gcb,'f16UpperLimit_Q');
      |     f16LowerLimit_Q_bkup=get_param(gcb,'f16LowerLimit_Q');
      |     u16NShift_bkup=get_param(gcb,'u16NShift');
      |     intmethod=get_param(gcb,'intmethod');
      |     if0=Simulink.data.evalinGlobal(bdroot,get_param(gcb,'if0'));
      |     iksi=Simulink.data.evalinGlobal(bdroot,get_param(gcb,'iksi'));
      |     Ld=Simulink.data.evalinGlobal(bdroot,get_param(gcb,'Ld'));
      |     Lq=Simulink.data.evalinGlobal(bdroot,get_param(gcb,'Lq'));
      |     Rs=Simulink.data.evalinGlobal(bdroot,get_param(gcb,'Rs'));
      |     mechspeed=Simulink.data.evalinGlobal(bdroot,get_param(gcb,'mechspeed'));
      |     polepairs=Simulink.data.evalinGlobal(bdroot,get_param(gcb,'polepairs'));
      |     uscale=Simulink.data.evalinGlobal(bdroot,get_param(gcb,'uscale'));
      |     escale=Simulink.data.evalinGlobal(bdroot,get_param(gcb,'escale'));
      |     iscale=Simulink.data.evalinGlobal(bdroot,get_param(gcb,'iscale'));
      |     if (if0<=0)
      |       warning('Natural frequency f0 must be positive.');
      |     end
      |     if (iksi<=0)
      |       warning('Current loop attenuation must be positive.');
      |     end
      |     if (iksi>1)
      |       warning('Current loop attenuation must not exceed 1.');
      |     end
      |     if (Ld<=0)
      |       warning('Inductance Ld must be positive.');
      |     end
      |     if (Lq<=0)
      |       warning('Inductance Lq must be positive.');
      |     end
      |     if (Rs<0)
      |       warning('Resistance Rs must be non-negative.');
      |     end
      |     if (mechspeed<=0)
      |       warning('Max. speed must be positive.');
      |     end
      |     if (polepairs<1)
      |       warning('Number of pole pairs must be a natural number (1, 2, 3, ...).');
      |     end
      |     if (round(polepairs)~=polepairs)
      |       warning('Number of pole pairs must be a natural number (1, 2, 3, ...).');
      |     end
      |     if (uscale<=0)
      |       warning('U_max must be positive.');
      |     end
      |     if (uscale>escale)
      |       warning('U_max must not exceed E_max');
      |     end
      |     if (iscale<=0)
      |       warning('I_max must be positive.');
      |     end
      |     if (escale<=0)
      |       warning('E_max must be positive.');
      |     end
      |     w0=6.283185307179586*if0;
      |     pgain=2.0*iksi*w0*Ld-Rs;
      |     igain=w0*w0*Ld;
      |     if strcmp(intmethod,'Forward Rectangular')
      |       cc1=pgain;
      |       cc2=-pgain+igain*SampleTime;
      |     else
      |       if strcmp(intmethod,'Backward Rectangular')
      |         cc1=pgain+igain*SampleTime;
      |         cc2=-pgain;
      |       else
      |         cc1=pgain+igain*SampleTime*0.5;
      |         cc2=-pgain+igain*SampleTime*0.5;
      |       end
      |     end
      |     cc1f=cc1*iscale/escale;
      |     cc2f=cc2*iscale/escale;
      |     u16NShift=ceil(log2(abs(cc1f)));
      |     tmpsh=ceil(log2(abs(cc2f)));
      |     if u16NShift<tmpsh
      |       u16NShift=tmpsh;
      |     end
      |     if u16NShift<0
      |       u16NShift=0;
      |     end
      |     if u16NShift>15
      |       u16NShift=15;
      |       warning(['Parameter u16NShift of ' gcb ' exceeds the fixed-point range.']);
      |     end
      |     f16CC1sc_D=round(cc1f*2^(-u16NShift)*2^15);
      |     if f16CC1sc_D>2^15-1
      |       f16CC1sc_D=2^15-1;
      |       warning(['Parameter f16CC1sc_D of ' gcb ' exceeds the fixed-point range.']);
      |     end
      |     if f16CC1sc_D<-2^15
      |       f16CC1sc_D=-2^15;
      |       warning(['Parameter f16CC1sc_D of ' gcb ' exceeds the fixed-point range.']);
      |     end
      |     f16CC2sc_D=round(cc2f*2^(-u16NShift)*2^15);
      |     if f16CC2sc_D>2^15-1
      |       f16CC2sc_D=2^15-1;
      |       warning(['Parameter f16CC2sc_D of ' gcb ' exceeds the fixed-point range.']);
      |     end
      |     if f16CC2sc_D<-2^15
      |       f16CC2sc_D=-2^15;
      |       warning(['Parameter f16CC2sc_D of ' gcb ' exceeds the fixed-point range.']);
      |     end
      |     f16LowerLimit_D=-32768;
      |     f16UpperLimit_D=32767;
      |     f16CC1sc_Q=f16CC1sc_D;
      |     f16CC2sc_Q=f16CC2sc_D;
      |     f16LowerLimit_Q=f16LowerLimit_D;
      |     f16UpperLimit_Q=f16UpperLimit_D;
      |     wmax=polepairs*mechspeed*1.047197551196598e-01;
      |     igainsc=(2.0*Ld-SampleTime*Rs)/(2.0*Ld+SampleTime*Rs);
      |     ugainsc=SampleTime/(2.0*Ld+SampleTime*Rs)*uscale/iscale;
      |     wigainsc=SampleTime*Lq/(2.0*Ld+SampleTime*Rs)*wmax;
      |     egainsc=SampleTime/(2.0*Ld+SampleTime*Rs)*escale/iscale;
      |     maxgain=max(abs([ugainsc,wigainsc,egainsc]));
      |     s16Shift=ceil(log2(abs(maxgain)));
      |     if s16Shift<-15
      |       s16Shift=-15;
      |     end
      |     if s16Shift>15
      |       s16Shift=15;
      |       warning(['Parameter s16Shift of ' gcb ' exceeds the fixed-point range.']);
      |     end
      |     f16IGain=round(igainsc*2^15);
      |     if f16IGain>2^15-1
      |       f16IGain=2^15-1;
      |       warning(['Parameter f16IGain of ' gcb ' exceeds the fixed-point range.']);
      |     end
      |     if f16IGain<-2^15
      |       f16IGain=-2^15;
      |       warning(['Parameter f16IGain of ' gcb ' exceeds the fixed-point range.']);
      |     end
      |     f16UGain=round(ugainsc*2^(-s16Shift)*2^15);
      |     if f16UGain>2^15-1
      |       f16UGain=2^15-1;
      |       warning(['Parameter f16UGain of ' gcb ' exceeds the fixed-point range.']);
      |     end
      |     if f16UGain<-2^15
      |       f16UGain=-2^15;
      |       warning(['Parameter f16UGain of ' gcb ' exceeds the fixed-point range.']);
      |     end
      |     f16WIGain=round(wigainsc*2^(-s16Shift)*2^15);
      |     if f16WIGain>2^15-1
      |       f16WIGain=2^15-1;
      |       warning(['Parameter f16WIGain of ' gcb ' exceeds the fixed-point range.']);
      |     end
      |     if f16WIGain<-2^15
      |       f16WIGain=-2^15;
      |       warning(['Parameter f16WIGain of ' gcb ' exceeds the fixed-point range.']);
      |     end
      |     f16EGain=round(egainsc*2^(-s16Shift)*2^15);
      |     if f16EGain>2^15-1
      |       f16EGain=2^15-1;
      |       warning(['Parameter f16EGain of ' gcb ' exceeds the fixed-point range.']);
      |     end
      |     if f16EGain<-2^15
      |       f16EGain=-2^15;
      |       warning(['Parameter f16EGain of ' gcb ' exceeds the fixed-point range.']);
      |     end
      |     if isnan(f16IGain)
      |       if ~strcmp(f16IGain_bkup,'0')
      |         set_param(gcb,'f16IGain','0');
      |       end
      |     else
      |       tmps=num2str(f16IGain);
      |       if ~strcmp(f16IGain_bkup,tmps)
      |         set_param(gcb,'f16IGain',tmps);
      |       end
      |     end
      |     if isnan(f16UGain)
      |       if ~strcmp(f16UGain_bkup,'0')
      |         set_param(gcb,'f16UGain','0');
      |       end
      |     else
      |       tmps=num2str(f16UGain);
      |       if ~strcmp(f16UGain_bkup,tmps)
      |         set_param(gcb,'f16UGain',tmps);
      |       end
      |     end
      |     if isnan(f16WIGain)
      |       if ~strcmp(f16WIGain_bkup,'0')
      |         set_param(gcb,'f16WIGain','0');
      |       end
      |     else
      |       tmps=num2str(f16WIGain);
      |       if ~strcmp(f16WIGain_bkup,tmps)
      |         set_param(gcb,'f16WIGain',tmps);
      |       end
      |     end
      |     if isnan(f16EGain)
      |       if ~strcmp(f16EGain_bkup,'0')
      |         set_param(gcb,'f16EGain','0');
      |       end
      |     else
      |       tmps=num2str(f16EGain);
      |       if ~strcmp(f16EGain_bkup,tmps)
      |         set_param(gcb,'f16EGain',tmps);
      |       end
      |     end
      |     if isnan(s16Shift)
      |       if ~strcmp(s16Shift_bkup,'0')
      |         set_param(gcb,'s16Shift','0');
      |       end
      |     else
      |       tmps=num2str(s16Shift);
      |       if ~strcmp(s16Shift_bkup,tmps)
      |         set_param(gcb,'s16Shift',tmps);
      |       end
      |     end
      |     if isnan(f16CC1sc_D)
      |       if ~strcmp(f16CC1sc_D_bkup,'0')
      |         set_param(gcb,'f16CC1sc_D','0');
      |       end
      |     else
      |       tmps=num2str(f16CC1sc_D);
      |       if ~strcmp(f16CC1sc_D_bkup,tmps)
      |         set_param(gcb,'f16CC1sc_D',tmps);
      |       end
      |     end
      |     if isnan(f16CC2sc_D)
      |       if ~strcmp(f16CC2sc_D_bkup,'0')
      |         set_param(gcb,'f16CC2sc_D','0');
      |       end
      |     else
      |       tmps=num2str(f16CC2sc_D);
      |       if ~strcmp(f16CC2sc_D_bkup,tmps)
      |         set_param(gcb,'f16CC2sc_D',tmps);
      |       end
      |     end
      |     if isnan(f16UpperLimit_D)
      |       if ~strcmp(f16UpperLimit_D_bkup,'0')
      |         set_param(gcb,'f16UpperLimit_D','0');
      |       end
      |     else
      |       tmps=num2str(f16UpperLimit_D);
      |       if ~strcmp(f16UpperLimit_D_bkup,tmps)
      |         set_param(gcb,'f16UpperLimit_D',tmps);
      |       end
      |     end
      |     if isnan(f16LowerLimit_D)
      |       if ~strcmp(f16LowerLimit_D_bkup,'0')
      |         set_param(gcb,'f16LowerLimit_D','0');
      |       end
      |     else
      |       tmps=num2str(f16LowerLimit_D);
      |       if ~strcmp(f16LowerLimit_D_bkup,tmps)
      |         set_param(gcb,'f16LowerLimit_D',tmps);
      |       end
      |     end
      |     if isnan(f16CC1sc_Q)
      |       if ~strcmp(f16CC1sc_Q_bkup,'0')
      |         set_param(gcb,'f16CC1sc_Q','0');
      |       end
      |     else
      |       tmps=num2str(f16CC1sc_Q);
      |       if ~strcmp(f16CC1sc_Q_bkup,tmps)
      |         set_param(gcb,'f16CC1sc_Q',tmps);
      |       end
      |     end
      |     if isnan(f16CC2sc_Q)
      |       if ~strcmp(f16CC2sc_Q_bkup,'0')
      |         set_param(gcb,'f16CC2sc_Q','0');
      |       end
      |     else
      |       tmps=num2str(f16CC2sc_Q);
      |       if ~strcmp(f16CC2sc_Q_bkup,tmps)
      |         set_param(gcb,'f16CC2sc_Q',tmps);
      |       end
      |     end
      |     if isnan(f16UpperLimit_Q)
      |       if ~strcmp(f16UpperLimit_Q_bkup,'0')
      |         set_param(gcb,'f16UpperLimit_Q','0');
      |       end
      |     else
      |       tmps=num2str(f16UpperLimit_Q);
      |       if ~strcmp(f16UpperLimit_Q_bkup,tmps)
      |         set_param(gcb,'f16UpperLimit_Q',tmps);
      |       end
      |     end
      |     if isnan(f16LowerLimit_Q)
      |       if ~strcmp(f16LowerLimit_Q_bkup,'0')
      |         set_param(gcb,'f16LowerLimit_Q','0');
      |       end
      |     else
      |       tmps=num2str(f16LowerLimit_Q);
      |       if ~strcmp(f16LowerLimit_Q_bkup,tmps)
      |         set_param(gcb,'f16LowerLimit_Q',tmps);
      |       end
      |     end
      |     if isnan(u16NShift)
      |       if ~strcmp(u16NShift_bkup,'0')
      |         set_param(gcb,'u16NShift','0');
      |       end
      |     else
      |       tmps=num2str(u16NShift);
      |       if ~strcmp(u16NShift_bkup,tmps)
      |         set_param(gcb,'u16NShift',tmps);
      |       end
      |     end
      |   end
      | end
      mask TypeOptions intmethod: Forward Rectangular | Backward Rectangular | Trapezoidal
      mask Callback intmethod:
      | autoCalcEn=get_param(gcb,'autoCalcEn');
      | if strcmp(autoCalcEn,'on')
      |   SampleTime=Simulink.data.evalinGlobal(bdroot,get_param(gcb,'SampleTime'));
      |   if (SampleTime==-1)
      |     SampleTime=str2double(get_param(gcb,'SampleTime_1'));
      |   end
      |   f16IGain_bkup=get_param(gcb,'f16IGain');
      |   f16UGain_bkup=get_param(gcb,'f16UGain');
      |   f16WIGain_bkup=get_param(gcb,'f16WIGain');
      |   f16EGain_bkup=get_param(gcb,'f16EGain');
      |   s16Shift_bkup=get_param(gcb,'s16Shift');
      |   f16CC1sc_D_bkup=get_param(gcb,'f16CC1sc_D');
      |   f16CC2sc_D_bkup=get_param(gcb,'f16CC2sc_D');
      |   f16UpperLimit_D_bkup=get_param(gcb,'f16UpperLimit_D');
      |   f16LowerLimit_D_bkup=get_param(gcb,'f16LowerLimit_D');
      |   f16CC1sc_Q_bkup=get_param(gcb,'f16CC1sc_Q');
      |   f16CC2sc_Q_bkup=get_param(gcb,'f16CC2sc_Q');
      |   f16UpperLimit_Q_bkup=get_param(gcb,'f16UpperLimit_Q');
      |   f16LowerLimit_Q_bkup=get_param(gcb,'f16LowerLimit_Q');
      |   u16NShift_bkup=get_param(gcb,'u16NShift');
      |   intmethod=get_param(gcb,'intmethod');
      |   if0=Simulink.data.evalinGlobal(bdroot,get_param(gcb,'if0'));
      |   iksi=Simulink.data.evalinGlobal(bdroot,get_param(gcb,'iksi'));
      |   Ld=Simulink.data.evalinGlobal(bdroot,get_param(gcb,'Ld'));
      |   Lq=Simulink.data.evalinGlobal(bdroot,get_param(gcb,'Lq'));
      |   Rs=Simulink.data.evalinGlobal(bdroot,get_param(gcb,'Rs'));
      |   mechspeed=Simulink.data.evalinGlobal(bdroot,get_param(gcb,'mechspeed'));
      |   polepairs=Simulink.data.evalinGlobal(bdroot,get_param(gcb,'polepairs'));
      |   uscale=Simulink.data.evalinGlobal(bdroot,get_param(gcb,'uscale'));
      |   escale=Simulink.data.evalinGlobal(bdroot,get_param(gcb,'escale'));
      |   iscale=Simulink.data.evalinGlobal(bdroot,get_param(gcb,'iscale'));
      |   if (if0<=0)
      |     warning('Natural frequency f0 must be positive.');
      |   end
      |   if (iksi<=0)
      |     warning('Current loop attenuation must be positive.');
      |   end
      |   if (iksi>1)
      |     warning('Current loop attenuation must not exceed 1.');
      |   end
      |   if (Ld<=0)
      |     warning('Inductance Ld must be positive.');
      |   end
      |   if (Lq<=0)
      |     warning('Inductance Lq must be positive.');
      |   end
      |   if (Rs<0)
      |     warning('Resistance Rs must be non-negative.');
      |   end
      |   if (mechspeed<=0)
      |     warning('Max. speed must be positive.');
      |   end
      |   if (polepairs<1)
      |     warning('Number of pole pairs must be a natural number (1, 2, 3, ...).');
      |   end
      |   if (round(polepairs)~=polepairs)
      |     warning('Number of pole pairs must be a natural number (1, 2, 3, ...).');
      |   end
      |   if (uscale<=0)
      |     warning('U_max must be positive.');
      |   end
      |   if (uscale>escale)
      |     warning('U_max must not exceed E_max');
      |   end
      |   if (iscale<=0)
      |     warning('I_max must be positive.');
      |   end
      |   if (escale<=0)
      |     warning('E_max must be positive.');
      |   end
      |   w0=6.283185307179586*if0;
      |   pgain=2.0*iksi*w0*Ld-Rs;
      |   igain=w0*w0*Ld;
      |   if strcmp(intmethod,'Forward Rectangular')
      |     cc1=pgain;
      |     cc2=-pgain+igain*SampleTime;
      |   else
      |     if strcmp(intmethod,'Backward Rectangular')
      |       cc1=pgain+igain*SampleTime;
      |       cc2=-pgain;
      |     else
      |       cc1=pgain+igain*SampleTime*0.5;
      |       cc2=-pgain+igain*SampleTime*0.5;
      |     end
      |   end
      |   cc1f=cc1*iscale/escale;
      |   cc2f=cc2*iscale/escale;
      |   u16NShift=ceil(log2(abs(cc1f)));
      |   tmpsh=ceil(log2(abs(cc2f)));
      |   if u16NShift<tmpsh
      |     u16NShift=tmpsh;
      |   end
      |   if u16NShift<0
      |     u16NShift=0;
      |   end
      |   if u16NShift>15
      |     u16NShift=15;
      |     warning(['Parameter u16NShift of ' gcb ' exceeds the fixed-point range.']);
      |   end
      |   f16CC1sc_D=round(cc1f*2^(-u16NShift)*2^15);
      |   if f16CC1sc_D>2^15-1
      |     f16CC1sc_D=2^15-1;
      |     warning(['Parameter f16CC1sc_D of ' gcb ' exceeds the fixed-point range.']);
      |   end
      |   if f16CC1sc_D<-2^15
      |     f16CC1sc_D=-2^15;
      |     warning(['Parameter f16CC1sc_D of ' gcb ' exceeds the fixed-point range.']);
      |   end
      |   f16CC2sc_D=round(cc2f*2^(-u16NShift)*2^15);
      |   if f16CC2sc_D>2^15-1
      |     f16CC2sc_D=2^15-1;
      |     warning(['Parameter f16CC2sc_D of ' gcb ' exceeds the fixed-point range.']);
      |   end
      |   if f16CC2sc_D<-2^15
      |     f16CC2sc_D=-2^15;
      |     warning(['Parameter f16CC2sc_D of ' gcb ' exceeds the fixed-point range.']);
      |   end
      |   f16LowerLimit_D=-32768;
      |   f16UpperLimit_D=32767;
      |   f16CC1sc_Q=f16CC1sc_D;
      |   f16CC2sc_Q=f16CC2sc_D;
      |   f16LowerLimit_Q=f16LowerLimit_D;
      |   f16UpperLimit_Q=f16UpperLimit_D;
      |   wmax=polepairs*mechspeed*1.047197551196598e-01;
      |   igainsc=(2.0*Ld-SampleTime*Rs)/(2.0*Ld+SampleTime*Rs);
      |   ugainsc=SampleTime/(2.0*Ld+SampleTime*Rs)*uscale/iscale;
      |   wigainsc=SampleTime*Lq/(2.0*Ld+SampleTime*Rs)*wmax;
      |   egainsc=SampleTime/(2.0*Ld+SampleTime*Rs)*escale/iscale;
      |   maxgain=max(abs([ugainsc,wigainsc,egainsc]));
      |   s16Shift=ceil(log2(abs(maxgain)));
      |   if s16Shift<-15
      |     s16Shift=-15;
      |   end
      |   if s16Shift>15
      |     s16Shift=15;
      |     warning(['Parameter s16Shift of ' gcb ' exceeds the fixed-point range.']);
      |   end
      |   f16IGain=round(igainsc*2^15);
      |   if f16IGain>2^15-1
      |     f16IGain=2^15-1;
      |     warning(['Parameter f16IGain of ' gcb ' exceeds the fixed-point range.']);
      |   end
      |   if f16IGain<-2^15
      |     f16IGain=-2^15;
      |     warning(['Parameter f16IGain of ' gcb ' exceeds the fixed-point range.']);
      |   end
      |   f16UGain=round(ugainsc*2^(-s16Shift)*2^15);
      |   if f16UGain>2^15-1
      |     f16UGain=2^15-1;
      |     warning(['Parameter f16UGain of ' gcb ' exceeds the fixed-point range.']);
      |   end
      |   if f16UGain<-2^15
      |     f16UGain=-2^15;
      |     warning(['Parameter f16UGain of ' gcb ' exceeds the fixed-point range.']);
      |   end
      |   f16WIGain=round(wigainsc*2^(-s16Shift)*2^15);
      |   if f16WIGain>2^15-1
      |     f16WIGain=2^15-1;
      |     warning(['Parameter f16WIGain of ' gcb ' exceeds the fixed-point range.']);
      |   end
      |   if f16WIGain<-2^15
      |     f16WIGain=-2^15;
      |     warning(['Parameter f16WIGain of ' gcb ' exceeds the fixed-point range.']);
      |   end
      |   f16EGain=round(egainsc*2^(-s16Shift)*2^15);
      |   if f16EGain>2^15-1
      |     f16EGain=2^15-1;
      |     warning(['Parameter f16EGain of ' gcb ' exceeds the fixed-point range.']);
      |   end
      |   if f16EGain<-2^15
      |     f16EGain=-2^15;
      |     warning(['Parameter f16EGain of ' gcb ' exceeds the fixed-point range.']);
      |   end
      |   if isnan(f16IGain)
      |     if ~strcmp(f16IGain_bkup,'0')
      |       set_param(gcb,'f16IGain','0');
      |     end
      |   else
      |     tmps=num2str(f16IGain);
      |     if ~strcmp(f16IGain_bkup,tmps)
      |       set_param(gcb,'f16IGain',tmps);
      |     end
      |   end
      |   if isnan(f16UGain)
      |     if ~strcmp(f16UGain_bkup,'0')
      |       set_param(gcb,'f16UGain','0');
      |     end
      |   else
      |     tmps=num2str(f16UGain);
      |     if ~strcmp(f16UGain_bkup,tmps)
      |       set_param(gcb,'f16UGain',tmps);
      |     end
      |   end
      |   if isnan(f16WIGain)
      |     if ~strcmp(f16WIGain_bkup,'0')
      |       set_param(gcb,'f16WIGain','0');
      |     end
      |   else
      |     tmps=num2str(f16WIGain);
      |     if ~strcmp(f16WIGain_bkup,tmps)
      |       set_param(gcb,'f16WIGain',tmps);
      |     end
      |   end
      |   if isnan(f16EGain)
      |     if ~strcmp(f16EGain_bkup,'0')
      |       set_param(gcb,'f16EGain','0');
      |     end
      |   else
      |     tmps=num2str(f16EGain);
      |     if ~strcmp(f16EGain_bkup,tmps)
      |       set_param(gcb,'f16EGain',tmps);
      |     end
      |   end
      |   if isnan(s16Shift)
      |     if ~strcmp(s16Shift_bkup,'0')
      |       set_param(gcb,'s16Shift','0');
      |     end
      |   else
      |     tmps=num2str(s16Shift);
      |     if ~strcmp(s16Shift_bkup,tmps)
      |       set_param(gcb,'s16Shift',tmps);
      |     end
      |   end
      |   if isnan(f16CC1sc_D)
      |     if ~strcmp(f16CC1sc_D_bkup,'0')
      |       set_param(gcb,'f16CC1sc_D','0');
      |     end
      |   else
      |     tmps=num2str(f16CC1sc_D);
      |     if ~strcmp(f16CC1sc_D_bkup,tmps)
      |       set_param(gcb,'f16CC1sc_D',tmps);
      |     end
      |   end
      |   if isnan(f16CC2sc_D)
      |     if ~strcmp(f16CC2sc_D_bkup,'0')
      |       set_param(gcb,'f16CC2sc_D','0');
      |     end
      |   else
      |     tmps=num2str(f16CC2sc_D);
      |     if ~strcmp(f16CC2sc_D_bkup,tmps)
      |       set_param(gcb,'f16CC2sc_D',tmps);
      |     end
      |   end
      |   if isnan(f16UpperLimit_D)
      |     if ~strcmp(f16UpperLimit_D_bkup,'0')
      |       set_param(gcb,'f16UpperLimit_D','0');
      |     end
      |   else
      |     tmps=num2str(f16UpperLimit_D);
      |     if ~strcmp(f16UpperLimit_D_bkup,tmps)
      |       set_param(gcb,'f16UpperLimit_D',tmps);
      |     end
      |   end
      |   if isnan(f16LowerLimit_D)
      |     if ~strcmp(f16LowerLimit_D_bkup,'0')
      |       set_param(gcb,'f16LowerLimit_D','0');
      |     end
      |   else
      |     tmps=num2str(f16LowerLimit_D);
      |     if ~strcmp(f16LowerLimit_D_bkup,tmps)
      |       set_param(gcb,'f16LowerLimit_D',tmps);
      |     end
      |   end
      |   if isnan(f16CC1sc_Q)
      |     if ~strcmp(f16CC1sc_Q_bkup,'0')
      |       set_param(gcb,'f16CC1sc_Q','0');
      |     end
      |   else
      |     tmps=num2str(f16CC1sc_Q);
      |     if ~strcmp(f16CC1sc_Q_bkup,tmps)
      |       set_param(gcb,'f16CC1sc_Q',tmps);
      |     end
      |   end
      |   if isnan(f16CC2sc_Q)
      |     if ~strcmp(f16CC2sc_Q_bkup,'0')
      |       set_param(gcb,'f16CC2sc_Q','0');
      |     end
      |   else
      |     tmps=num2str(f16CC2sc_Q);
      |     if ~strcmp(f16CC2sc_Q_bkup,tmps)
      |       set_param(gcb,'f16CC2sc_Q',tmps);
      |     end
      |   end
      |   if isnan(f16UpperLimit_Q)
      |     if ~strcmp(f16UpperLimit_Q_bkup,'0')
      |       set_param(gcb,'f16UpperLimit_Q','0');
      |     end
      |   else
      |     tmps=num2str(f16UpperLimit_Q);
      |     if ~strcmp(f16UpperLimit_Q_bkup,tmps)
      |       set_param(gcb,'f16UpperLimit_Q',tmps);
      |     end
      |   end
      |   if isnan(f16LowerLimit_Q)
      |     if ~strcmp(f16LowerLimit_Q_bkup,'0')
      |       set_param(gcb,'f16LowerLimit_Q','0');
      |     end
      |   else
      |     tmps=num2str(f16LowerLimit_Q);
      |     if ~strcmp(f16LowerLimit_Q_bkup,tmps)
      |       set_param(gcb,'f16LowerLimit_Q',tmps);
      |     end
      |   end
      |   if isnan(u16NShift)
      |     if ~strcmp(u16NShift_bkup,'0')
      |       set_param(gcb,'u16NShift','0');
      |     end
      |   else
      |     tmps=num2str(u16NShift);
      |     if ~strcmp(u16NShift_bkup,tmps)
      |       set_param(gcb,'u16NShift',tmps);
      |     end
      |   end
      | end
      mask Callback if0:
      | autoCalcEn=get_param(gcb,'autoCalcEn');
      | if strcmp(autoCalcEn,'on')
      |   SampleTime=Simulink.data.evalinGlobal(bdroot,get_param(gcb,'SampleTime'));
      |   if (SampleTime==-1)
      |     SampleTime=str2double(get_param(gcb,'SampleTime_1'));
      |   end
      |   f16IGain_bkup=get_param(gcb,'f16IGain');
      |   f16UGain_bkup=get_param(gcb,'f16UGain');
      |   f16WIGain_bkup=get_param(gcb,'f16WIGain');
      |   f16EGain_bkup=get_param(gcb,'f16EGain');
      |   s16Shift_bkup=get_param(gcb,'s16Shift');
      |   f16CC1sc_D_bkup=get_param(gcb,'f16CC1sc_D');
      |   f16CC2sc_D_bkup=get_param(gcb,'f16CC2sc_D');
      |   f16UpperLimit_D_bkup=get_param(gcb,'f16UpperLimit_D');
      |   f16LowerLimit_D_bkup=get_param(gcb,'f16LowerLimit_D');
      |   f16CC1sc_Q_bkup=get_param(gcb,'f16CC1sc_Q');
      |   f16CC2sc_Q_bkup=get_param(gcb,'f16CC2sc_Q');
      |   f16UpperLimit_Q_bkup=get_param(gcb,'f16UpperLimit_Q');
      |   f16LowerLimit_Q_bkup=get_param(gcb,'f16LowerLimit_Q');
      |   u16NShift_bkup=get_param(gcb,'u16NShift');
      |   intmethod=get_param(gcb,'intmethod');
      |   if0=Simulink.data.evalinGlobal(bdroot,get_param(gcb,'if0'));
      |   iksi=Simulink.data.evalinGlobal(bdroot,get_param(gcb,'iksi'));
      |   Ld=Simulink.data.evalinGlobal(bdroot,get_param(gcb,'Ld'));
      |   Lq=Simulink.data.evalinGlobal(bdroot,get_param(gcb,'Lq'));
      |   Rs=Simulink.data.evalinGlobal(bdroot,get_param(gcb,'Rs'));
      |   mechspeed=Simulink.data.evalinGlobal(bdroot,get_param(gcb,'mechspeed'));
      |   polepairs=Simulink.data.evalinGlobal(bdroot,get_param(gcb,'polepairs'));
      |   uscale=Simulink.data.evalinGlobal(bdroot,get_param(gcb,'uscale'));
      |   escale=Simulink.data.evalinGlobal(bdroot,get_param(gcb,'escale'));
      |   iscale=Simulink.data.evalinGlobal(bdroot,get_param(gcb,'iscale'));
      |   if (if0<=0)
      |     warning('Natural frequency f0 must be positive.');
      |   end
      |   if (iksi<=0)
      |     warning('Current loop attenuation must be positive.');
      |   end
      |   if (iksi>1)
      |     warning('Current loop attenuation must not exceed 1.');
      |   end
      |   if (Ld<=0)
      |     warning('Inductance Ld must be positive.');
      |   end
      |   if (Lq<=0)
      |     warning('Inductance Lq must be positive.');
      |   end
      |   if (Rs<0)
      |     warning('Resistance Rs must be non-negative.');
      |   end
      |   if (mechspeed<=0)
      |     warning('Max. speed must be positive.');
      |   end
      |   if (polepairs<1)
      |     warning('Number of pole pairs must be a natural number (1, 2, 3, ...).');
      |   end
      |   if (round(polepairs)~=polepairs)
      |     warning('Number of pole pairs must be a natural number (1, 2, 3, ...).');
      |   end
      |   if (uscale<=0)
      |     warning('U_max must be positive.');
      |   end
      |   if (uscale>escale)
      |     warning('U_max must not exceed E_max');
      |   end
      |   if (iscale<=0)
      |     warning('I_max must be positive.');
      |   end
      |   if (escale<=0)
      |     warning('E_max must be positive.');
      |   end
      |   w0=6.283185307179586*if0;
      |   pgain=2.0*iksi*w0*Ld-Rs;
      |   igain=w0*w0*Ld;
      |   if strcmp(intmethod,'Forward Rectangular')
      |     cc1=pgain;
      |     cc2=-pgain+igain*SampleTime;
      |   else
      |     if strcmp(intmethod,'Backward Rectangular')
      |       cc1=pgain+igain*SampleTime;
      |       cc2=-pgain;
      |     else
      |       cc1=pgain+igain*SampleTime*0.5;
      |       cc2=-pgain+igain*SampleTime*0.5;
      |     end
      |   end
      |   cc1f=cc1*iscale/escale;
      |   cc2f=cc2*iscale/escale;
      |   u16NShift=ceil(log2(abs(cc1f)));
      |   tmpsh=ceil(log2(abs(cc2f)));
      |   if u16NShift<tmpsh
      |     u16NShift=tmpsh;
      |   end
      |   if u16NShift<0
      |     u16NShift=0;
      |   end
      |   if u16NShift>15
      |     u16NShift=15;
      |     warning(['Parameter u16NShift of ' gcb ' exceeds the fixed-point range.']);
      |   end
      |   f16CC1sc_D=round(cc1f*2^(-u16NShift)*2^15);
      |   if f16CC1sc_D>2^15-1
      |     f16CC1sc_D=2^15-1;
      |     warning(['Parameter f16CC1sc_D of ' gcb ' exceeds the fixed-point range.']);
      |   end
      |   if f16CC1sc_D<-2^15
      |     f16CC1sc_D=-2^15;
      |     warning(['Parameter f16CC1sc_D of ' gcb ' exceeds the fixed-point range.']);
      |   end
      |   f16CC2sc_D=round(cc2f*2^(-u16NShift)*2^15);
      |   if f16CC2sc_D>2^15-1
      |     f16CC2sc_D=2^15-1;
      |     warning(['Parameter f16CC2sc_D of ' gcb ' exceeds the fixed-point range.']);
      |   end
      |   if f16CC2sc_D<-2^15
      |     f16CC2sc_D=-2^15;
      |     warning(['Parameter f16CC2sc_D of ' gcb ' exceeds the fixed-point range.']);
      |   end
      |   f16LowerLimit_D=-32768;
      |   f16UpperLimit_D=32767;
      |   f16CC1sc_Q=f16CC1sc_D;
      |   f16CC2sc_Q=f16CC2sc_D;
      |   f16LowerLimit_Q=f16LowerLimit_D;
      |   f16UpperLimit_Q=f16UpperLimit_D;
      |   wmax=polepairs*mechspeed*1.047197551196598e-01;
      |   igainsc=(2.0*Ld-SampleTime*Rs)/(2.0*Ld+SampleTime*Rs);
      |   ugainsc=SampleTime/(2.0*Ld+SampleTime*Rs)*uscale/iscale;
      |   wigainsc=SampleTime*Lq/(2.0*Ld+SampleTime*Rs)*wmax;
      |   egainsc=SampleTime/(2.0*Ld+SampleTime*Rs)*escale/iscale;
      |   maxgain=max(abs([ugainsc,wigainsc,egainsc]));
      |   s16Shift=ceil(log2(abs(maxgain)));
      |   if s16Shift<-15
      |     s16Shift=-15;
      |   end
      |   if s16Shift>15
      |     s16Shift=15;
      |     warning(['Parameter s16Shift of ' gcb ' exceeds the fixed-point range.']);
      |   end
      |   f16IGain=round(igainsc*2^15);
      |   if f16IGain>2^15-1
      |     f16IGain=2^15-1;
      |     warning(['Parameter f16IGain of ' gcb ' exceeds the fixed-point range.']);
      |   end
      |   if f16IGain<-2^15
      |     f16IGain=-2^15;
      |     warning(['Parameter f16IGain of ' gcb ' exceeds the fixed-point range.']);
      |   end
      |   f16UGain=round(ugainsc*2^(-s16Shift)*2^15);
      |   if f16UGain>2^15-1
      |     f16UGain=2^15-1;
      |     warning(['Parameter f16UGain of ' gcb ' exceeds the fixed-point range.']);
      |   end
      |   if f16UGain<-2^15
      |     f16UGain=-2^15;
      |     warning(['Parameter f16UGain of ' gcb ' exceeds the fixed-point range.']);
      |   end
      |   f16WIGain=round(wigainsc*2^(-s16Shift)*2^15);
      |   if f16WIGain>2^15-1
      |     f16WIGain=2^15-1;
      |     warning(['Parameter f16WIGain of ' gcb ' exceeds the fixed-point range.']);
      |   end
      |   if f16WIGain<-2^15
      |     f16WIGain=-2^15;
      |     warning(['Parameter f16WIGain of ' gcb ' exceeds the fixed-point range.']);
      |   end
      |   f16EGain=round(egainsc*2^(-s16Shift)*2^15);
      |   if f16EGain>2^15-1
      |     f16EGain=2^15-1;
      |     warning(['Parameter f16EGain of ' gcb ' exceeds the fixed-point range.']);
      |   end
      |   if f16EGain<-2^15
      |     f16EGain=-2^15;
      |     warning(['Parameter f16EGain of ' gcb ' exceeds the fixed-point range.']);
      |   end
      |   if isnan(f16IGain)
      |     if ~strcmp(f16IGain_bkup,'0')
      |       set_param(gcb,'f16IGain','0');
      |     end
      |   else
      |     tmps=num2str(f16IGain);
      |     if ~strcmp(f16IGain_bkup,tmps)
      |       set_param(gcb,'f16IGain',tmps);
      |     end
      |   end
      |   if isnan(f16UGain)
      |     if ~strcmp(f16UGain_bkup,'0')
      |       set_param(gcb,'f16UGain','0');
      |     end
      |   else
      |     tmps=num2str(f16UGain);
      |     if ~strcmp(f16UGain_bkup,tmps)
      |       set_param(gcb,'f16UGain',tmps);
      |     end
      |   end
      |   if isnan(f16WIGain)
      |     if ~strcmp(f16WIGain_bkup,'0')
      |       set_param(gcb,'f16WIGain','0');
      |     end
      |   else
      |     tmps=num2str(f16WIGain);
      |     if ~strcmp(f16WIGain_bkup,tmps)
      |       set_param(gcb,'f16WIGain',tmps);
      |     end
      |   end
      |   if isnan(f16EGain)
      |     if ~strcmp(f16EGain_bkup,'0')
      |       set_param(gcb,'f16EGain','0');
      |     end
      |   else
      |     tmps=num2str(f16EGain);
      |     if ~strcmp(f16EGain_bkup,tmps)
      |       set_param(gcb,'f16EGain',tmps);
      |     end
      |   end
      |   if isnan(s16Shift)
      |     if ~strcmp(s16Shift_bkup,'0')
      |       set_param(gcb,'s16Shift','0');
      |     end
      |   else
      |     tmps=num2str(s16Shift);
      |     if ~strcmp(s16Shift_bkup,tmps)
      |       set_param(gcb,'s16Shift',tmps);
      |     end
      |   end
      |   if isnan(f16CC1sc_D)
      |     if ~strcmp(f16CC1sc_D_bkup,'0')
      |       set_param(gcb,'f16CC1sc_D','0');
      |     end
      |   else
      |     tmps=num2str(f16CC1sc_D);
      |     if ~strcmp(f16CC1sc_D_bkup,tmps)
      |       set_param(gcb,'f16CC1sc_D',tmps);
      |     end
      |   end
      |   if isnan(f16CC2sc_D)
      |     if ~strcmp(f16CC2sc_D_bkup,'0')
      |       set_param(gcb,'f16CC2sc_D','0');
      |     end
      |   else
      |     tmps=num2str(f16CC2sc_D);
      |     if ~strcmp(f16CC2sc_D_bkup,tmps)
      |       set_param(gcb,'f16CC2sc_D',tmps);
      |     end
      |   end
      |   if isnan(f16UpperLimit_D)
      |     if ~strcmp(f16UpperLimit_D_bkup,'0')
      |       set_param(gcb,'f16UpperLimit_D','0');
      |     end
      |   else
      |     tmps=num2str(f16UpperLimit_D);
      |     if ~strcmp(f16UpperLimit_D_bkup,tmps)
      |       set_param(gcb,'f16UpperLimit_D',tmps);
      |     end
      |   end
      |   if isnan(f16LowerLimit_D)
      |     if ~strcmp(f16LowerLimit_D_bkup,'0')
      |       set_param(gcb,'f16LowerLimit_D','0');
      |     end
      |   else
      |     tmps=num2str(f16LowerLimit_D);
      |     if ~strcmp(f16LowerLimit_D_bkup,tmps)
      |       set_param(gcb,'f16LowerLimit_D',tmps);
      |     end
      |   end
      |   if isnan(f16CC1sc_Q)
      |     if ~strcmp(f16CC1sc_Q_bkup,'0')
      |       set_param(gcb,'f16CC1sc_Q','0');
      |     end
      |   else
      |     tmps=num2str(f16CC1sc_Q);
      |     if ~strcmp(f16CC1sc_Q_bkup,tmps)
      |       set_param(gcb,'f16CC1sc_Q',tmps);
      |     end
      |   end
      |   if isnan(f16CC2sc_Q)
      |     if ~strcmp(f16CC2sc_Q_bkup,'0')
      |       set_param(gcb,'f16CC2sc_Q','0');
      |     end
      |   else
      |     tmps=num2str(f16CC2sc_Q);
      |     if ~strcmp(f16CC2sc_Q_bkup,tmps)
      |       set_param(gcb,'f16CC2sc_Q',tmps);
      |     end
      |   end
      |   if isnan(f16UpperLimit_Q)
      |     if ~strcmp(f16UpperLimit_Q_bkup,'0')
      |       set_param(gcb,'f16UpperLimit_Q','0');
      |     end
      |   else
      |     tmps=num2str(f16UpperLimit_Q);
      |     if ~strcmp(f16UpperLimit_Q_bkup,tmps)
      |       set_param(gcb,'f16UpperLimit_Q',tmps);
      |     end
      |   end
      |   if isnan(f16LowerLimit_Q)
      |     if ~strcmp(f16LowerLimit_Q_bkup,'0')
      |       set_param(gcb,'f16LowerLimit_Q','0');
      |     end
      |   else
      |     tmps=num2str(f16LowerLimit_Q);
      |     if ~strcmp(f16LowerLimit_Q_bkup,tmps)
      |       set_param(gcb,'f16LowerLimit_Q',tmps);
      |     end
      |   end
      |   if isnan(u16NShift)
      |     if ~strcmp(u16NShift_bkup,'0')
      |       set_param(gcb,'u16NShift','0');
      |     end
      |   else
      |     tmps=num2str(u16NShift);
      |     if ~strcmp(u16NShift_bkup,tmps)
      |       set_param(gcb,'u16NShift',tmps);
      |     end
      |   end
      | end
      mask Callback iksi:
      | autoCalcEn=get_param(gcb,'autoCalcEn');
      | if strcmp(autoCalcEn,'on')
      |   SampleTime=Simulink.data.evalinGlobal(bdroot,get_param(gcb,'SampleTime'));
      |   if (SampleTime==-1)
      |     SampleTime=str2double(get_param(gcb,'SampleTime_1'));
      |   end
      |   f16IGain_bkup=get_param(gcb,'f16IGain');
      |   f16UGain_bkup=get_param(gcb,'f16UGain');
      |   f16WIGain_bkup=get_param(gcb,'f16WIGain');
      |   f16EGain_bkup=get_param(gcb,'f16EGain');
      |   s16Shift_bkup=get_param(gcb,'s16Shift');
      |   f16CC1sc_D_bkup=get_param(gcb,'f16CC1sc_D');
      |   f16CC2sc_D_bkup=get_param(gcb,'f16CC2sc_D');
      |   f16UpperLimit_D_bkup=get_param(gcb,'f16UpperLimit_D');
      |   f16LowerLimit_D_bkup=get_param(gcb,'f16LowerLimit_D');
      |   f16CC1sc_Q_bkup=get_param(gcb,'f16CC1sc_Q');
      |   f16CC2sc_Q_bkup=get_param(gcb,'f16CC2sc_Q');
      |   f16UpperLimit_Q_bkup=get_param(gcb,'f16UpperLimit_Q');
      |   f16LowerLimit_Q_bkup=get_param(gcb,'f16LowerLimit_Q');
      |   u16NShift_bkup=get_param(gcb,'u16NShift');
      |   intmethod=get_param(gcb,'intmethod');
      |   if0=Simulink.data.evalinGlobal(bdroot,get_param(gcb,'if0'));
      |   iksi=Simulink.data.evalinGlobal(bdroot,get_param(gcb,'iksi'));
      |   Ld=Simulink.data.evalinGlobal(bdroot,get_param(gcb,'Ld'));
      |   Lq=Simulink.data.evalinGlobal(bdroot,get_param(gcb,'Lq'));
      |   Rs=Simulink.data.evalinGlobal(bdroot,get_param(gcb,'Rs'));
      |   mechspeed=Simulink.data.evalinGlobal(bdroot,get_param(gcb,'mechspeed'));
      |   polepairs=Simulink.data.evalinGlobal(bdroot,get_param(gcb,'polepairs'));
      |   uscale=Simulink.data.evalinGlobal(bdroot,get_param(gcb,'uscale'));
      |   escale=Simulink.data.evalinGlobal(bdroot,get_param(gcb,'escale'));
      |   iscale=Simulink.data.evalinGlobal(bdroot,get_param(gcb,'iscale'));
      |   if (if0<=0)
      |     warning('Natural frequency f0 must be positive.');
      |   end
      |   if (iksi<=0)
      |     warning('Current loop attenuation must be positive.');
      |   end
      |   if (iksi>1)
      |     warning('Current loop attenuation must not exceed 1.');
      |   end
      |   if (Ld<=0)
      |     warning('Inductance Ld must be positive.');
      |   end
      |   if (Lq<=0)
      |     warning('Inductance Lq must be positive.');
      |   end
      |   if (Rs<0)
      |     warning('Resistance Rs must be non-negative.');
      |   end
      |   if (mechspeed<=0)
      |     warning('Max. speed must be positive.');
      |   end
      |   if (polepairs<1)
      |     warning('Number of pole pairs must be a natural number (1, 2, 3, ...).');
      |   end
      |   if (round(polepairs)~=polepairs)
      |     warning('Number of pole pairs must be a natural number (1, 2, 3, ...).');
      |   end
      |   if (uscale<=0)
      |     warning('U_max must be positive.');
      |   end
      |   if (uscale>escale)
      |     warning('U_max must not exceed E_max');
      |   end
      |   if (iscale<=0)
      |     warning('I_max must be positive.');
      |   end
      |   if (escale<=0)
      |     warning('E_max must be positive.');
      |   end
      |   w0=6.283185307179586*if0;
      |   pgain=2.0*iksi*w0*Ld-Rs;
      |   igain=w0*w0*Ld;
      |   if strcmp(intmethod,'Forward Rectangular')
      |     cc1=pgain;
      |     cc2=-pgain+igain*SampleTime;
      |   else
      |     if strcmp(intmethod,'Backward Rectangular')
      |       cc1=pgain+igain*SampleTime;
      |       cc2=-pgain;
      |     else
      |       cc1=pgain+igain*SampleTime*0.5;
      |       cc2=-pgain+igain*SampleTime*0.5;
      |     end
      |   end
      |   cc1f=cc1*iscale/escale;
      |   cc2f=cc2*iscale/escale;
      |   u16NShift=ceil(log2(abs(cc1f)));
      |   tmpsh=ceil(log2(abs(cc2f)));
      |   if u16NShift<tmpsh
      |     u16NShift=tmpsh;
      |   end
      |   if u16NShift<0
      |     u16NShift=0;
      |   end
      |   if u16NShift>15
      |     u16NShift=15;
      |     warning(['Parameter u16NShift of ' gcb ' exceeds the fixed-point range.']);
      |   end
      |   f16CC1sc_D=round(cc1f*2^(-u16NShift)*2^15);
      |   if f16CC1sc_D>2^15-1
      |     f16CC1sc_D=2^15-1;
      |     warning(['Parameter f16CC1sc_D of ' gcb ' exceeds the fixed-point range.']);
      |   end
      |   if f16CC1sc_D<-2^15
      |     f16CC1sc_D=-2^15;
      |     warning(['Parameter f16CC1sc_D of ' gcb ' exceeds the fixed-point range.']);
      |   end
      |   f16CC2sc_D=round(cc2f*2^(-u16NShift)*2^15);
      |   if f16CC2sc_D>2^15-1
      |     f16CC2sc_D=2^15-1;
      |     warning(['Parameter f16CC2sc_D of ' gcb ' exceeds the fixed-point range.']);
      |   end
      |   if f16CC2sc_D<-2^15
      |     f16CC2sc_D=-2^15;
      |     warning(['Parameter f16CC2sc_D of ' gcb ' exceeds the fixed-point range.']);
      |   end
      |   f16LowerLimit_D=-32768;
      |   f16UpperLimit_D=32767;
      |   f16CC1sc_Q=f16CC1sc_D;
      |   f16CC2sc_Q=f16CC2sc_D;
      |   f16LowerLimit_Q=f16LowerLimit_D;
      |   f16UpperLimit_Q=f16UpperLimit_D;
      |   wmax=polepairs*mechspeed*1.047197551196598e-01;
      |   igainsc=(2.0*Ld-SampleTime*Rs)/(2.0*Ld+SampleTime*Rs);
      |   ugainsc=SampleTime/(2.0*Ld+SampleTime*Rs)*uscale/iscale;
      |   wigainsc=SampleTime*Lq/(2.0*Ld+SampleTime*Rs)*wmax;
      |   egainsc=SampleTime/(2.0*Ld+SampleTime*Rs)*escale/iscale;
      |   maxgain=max(abs([ugainsc,wigainsc,egainsc]));
      |   s16Shift=ceil(log2(abs(maxgain)));
      |   if s16Shift<-15
      |     s16Shift=-15;
      |   end
      |   if s16Shift>15
      |     s16Shift=15;
      |     warning(['Parameter s16Shift of ' gcb ' exceeds the fixed-point range.']);
      |   end
      |   f16IGain=round(igainsc*2^15);
      |   if f16IGain>2^15-1
      |     f16IGain=2^15-1;
      |     warning(['Parameter f16IGain of ' gcb ' exceeds the fixed-point range.']);
      |   end
      |   if f16IGain<-2^15
      |     f16IGain=-2^15;
      |     warning(['Parameter f16IGain of ' gcb ' exceeds the fixed-point range.']);
      |   end
      |   f16UGain=round(ugainsc*2^(-s16Shift)*2^15);
      |   if f16UGain>2^15-1
      |     f16UGain=2^15-1;
      |     warning(['Parameter f16UGain of ' gcb ' exceeds the fixed-point range.']);
      |   end
      |   if f16UGain<-2^15
      |     f16UGain=-2^15;
      |     warning(['Parameter f16UGain of ' gcb ' exceeds the fixed-point range.']);
      |   end
      |   f16WIGain=round(wigainsc*2^(-s16Shift)*2^15);
      |   if f16WIGain>2^15-1
      |     f16WIGain=2^15-1;
      |     warning(['Parameter f16WIGain of ' gcb ' exceeds the fixed-point range.']);
      |   end
      |   if f16WIGain<-2^15
      |     f16WIGain=-2^15;
      |     warning(['Parameter f16WIGain of ' gcb ' exceeds the fixed-point range.']);
      |   end
      |   f16EGain=round(egainsc*2^(-s16Shift)*2^15);
      |   if f16EGain>2^15-1
      |     f16EGain=2^15-1;
      |     warning(['Parameter f16EGain of ' gcb ' exceeds the fixed-point range.']);
      |   end
      |   if f16EGain<-2^15
      |     f16EGain=-2^15;
      |     warning(['Parameter f16EGain of ' gcb ' exceeds the fixed-point range.']);
      |   end
      |   if isnan(f16IGain)
      |     if ~strcmp(f16IGain_bkup,'0')
      |       set_param(gcb,'f16IGain','0');
      |     end
      |   else
      |     tmps=num2str(f16IGain);
      |     if ~strcmp(f16IGain_bkup,tmps)
      |       set_param(gcb,'f16IGain',tmps);
      |     end
      |   end
      |   if isnan(f16UGain)
      |     if ~strcmp(f16UGain_bkup,'0')
      |       set_param(gcb,'f16UGain','0');
      |     end
      |   else
      |     tmps=num2str(f16UGain);
      |     if ~strcmp(f16UGain_bkup,tmps)
      |       set_param(gcb,'f16UGain',tmps);
      |     end
      |   end
      |   if isnan(f16WIGain)
      |     if ~strcmp(f16WIGain_bkup,'0')
      |       set_param(gcb,'f16WIGain','0');
      |     end
      |   else
      |     tmps=num2str(f16WIGain);
      |     if ~strcmp(f16WIGain_bkup,tmps)
      |       set_param(gcb,'f16WIGain',tmps);
      |     end
      |   end
      |   if isnan(f16EGain)
      |     if ~strcmp(f16EGain_bkup,'0')
      |       set_param(gcb,'f16EGain','0');
      |     end
      |   else
      |     tmps=num2str(f16EGain);
      |     if ~strcmp(f16EGain_bkup,tmps)
      |       set_param(gcb,'f16EGain',tmps);
      |     end
      |   end
      |   if isnan(s16Shift)
      |     if ~strcmp(s16Shift_bkup,'0')
      |       set_param(gcb,'s16Shift','0');
      |     end
      |   else
      |     tmps=num2str(s16Shift);
      |     if ~strcmp(s16Shift_bkup,tmps)
      |       set_param(gcb,'s16Shift',tmps);
      |     end
      |   end
      |   if isnan(f16CC1sc_D)
      |     if ~strcmp(f16CC1sc_D_bkup,'0')
      |       set_param(gcb,'f16CC1sc_D','0');
      |     end
      |   else
      |     tmps=num2str(f16CC1sc_D);
      |     if ~strcmp(f16CC1sc_D_bkup,tmps)
      |       set_param(gcb,'f16CC1sc_D',tmps);
      |     end
      |   end
      |   if isnan(f16CC2sc_D)
      |     if ~strcmp(f16CC2sc_D_bkup,'0')
      |       set_param(gcb,'f16CC2sc_D','0');
      |     end
      |   else
      |     tmps=num2str(f16CC2sc_D);
      |     if ~strcmp(f16CC2sc_D_bkup,tmps)
      |       set_param(gcb,'f16CC2sc_D',tmps);
      |     end
      |   end
      |   if isnan(f16UpperLimit_D)
      |     if ~strcmp(f16UpperLimit_D_bkup,'0')
      |       set_param(gcb,'f16UpperLimit_D','0');
      |     end
      |   else
      |     tmps=num2str(f16UpperLimit_D);
      |     if ~strcmp(f16UpperLimit_D_bkup,tmps)
      |       set_param(gcb,'f16UpperLimit_D',tmps);
      |     end
      |   end
      |   if isnan(f16LowerLimit_D)
      |     if ~strcmp(f16LowerLimit_D_bkup,'0')
      |       set_param(gcb,'f16LowerLimit_D','0');
      |     end
      |   else
      |     tmps=num2str(f16LowerLimit_D);
      |     if ~strcmp(f16LowerLimit_D_bkup,tmps)
      |       set_param(gcb,'f16LowerLimit_D',tmps);
      |     end
      |   end
      |   if isnan(f16CC1sc_Q)
      |     if ~strcmp(f16CC1sc_Q_bkup,'0')
      |       set_param(gcb,'f16CC1sc_Q','0');
      |     end
      |   else
      |     tmps=num2str(f16CC1sc_Q);
      |     if ~strcmp(f16CC1sc_Q_bkup,tmps)
      |       set_param(gcb,'f16CC1sc_Q',tmps);
      |     end
      |   end
      |   if isnan(f16CC2sc_Q)
      |     if ~strcmp(f16CC2sc_Q_bkup,'0')
      |       set_param(gcb,'f16CC2sc_Q','0');
      |     end
      |   else
      |     tmps=num2str(f16CC2sc_Q);
      |     if ~strcmp(f16CC2sc_Q_bkup,tmps)
      |       set_param(gcb,'f16CC2sc_Q',tmps);
      |     end
      |   end
      |   if isnan(f16UpperLimit_Q)
      |     if ~strcmp(f16UpperLimit_Q_bkup,'0')
      |       set_param(gcb,'f16UpperLimit_Q','0');
      |     end
      |   else
      |     tmps=num2str(f16UpperLimit_Q);
      |     if ~strcmp(f16UpperLimit_Q_bkup,tmps)
      |       set_param(gcb,'f16UpperLimit_Q',tmps);
      |     end
      |   end
      |   if isnan(f16LowerLimit_Q)
      |     if ~strcmp(f16LowerLimit_Q_bkup,'0')
      |       set_param(gcb,'f16LowerLimit_Q','0');
      |     end
      |   else
      |     tmps=num2str(f16LowerLimit_Q);
      |     if ~strcmp(f16LowerLimit_Q_bkup,tmps)
      |       set_param(gcb,'f16LowerLimit_Q',tmps);
      |     end
      |   end
      |   if isnan(u16NShift)
      |     if ~strcmp(u16NShift_bkup,'0')
      |       set_param(gcb,'u16NShift','0');
      |     end
      |   else
      |     tmps=num2str(u16NShift);
      |     if ~strcmp(u16NShift_bkup,tmps)
      |       set_param(gcb,'u16NShift',tmps);
      |     end
      |   end
      | end
      mask Callback Ld:
      | autoCalcEn=get_param(gcb,'autoCalcEn');
      | if strcmp(autoCalcEn,'on')
      |   SampleTime=Simulink.data.evalinGlobal(bdroot,get_param(gcb,'SampleTime'));
      |   if (SampleTime==-1)
      |     SampleTime=str2double(get_param(gcb,'SampleTime_1'));
      |   end
      |   f16IGain_bkup=get_param(gcb,'f16IGain');
      |   f16UGain_bkup=get_param(gcb,'f16UGain');
      |   f16WIGain_bkup=get_param(gcb,'f16WIGain');
      |   f16EGain_bkup=get_param(gcb,'f16EGain');
      |   s16Shift_bkup=get_param(gcb,'s16Shift');
      |   f16CC1sc_D_bkup=get_param(gcb,'f16CC1sc_D');
      |   f16CC2sc_D_bkup=get_param(gcb,'f16CC2sc_D');
      |   f16UpperLimit_D_bkup=get_param(gcb,'f16UpperLimit_D');
      |   f16LowerLimit_D_bkup=get_param(gcb,'f16LowerLimit_D');
      |   f16CC1sc_Q_bkup=get_param(gcb,'f16CC1sc_Q');
      |   f16CC2sc_Q_bkup=get_param(gcb,'f16CC2sc_Q');
      |   f16UpperLimit_Q_bkup=get_param(gcb,'f16UpperLimit_Q');
      |   f16LowerLimit_Q_bkup=get_param(gcb,'f16LowerLimit_Q');
      |   u16NShift_bkup=get_param(gcb,'u16NShift');
      |   intmethod=get_param(gcb,'intmethod');
      |   if0=Simulink.data.evalinGlobal(bdroot,get_param(gcb,'if0'));
      |   iksi=Simulink.data.evalinGlobal(bdroot,get_param(gcb,'iksi'));
      |   Ld=Simulink.data.evalinGlobal(bdroot,get_param(gcb,'Ld'));
      |   Lq=Simulink.data.evalinGlobal(bdroot,get_param(gcb,'Lq'));
      |   Rs=Simulink.data.evalinGlobal(bdroot,get_param(gcb,'Rs'));
      |   mechspeed=Simulink.data.evalinGlobal(bdroot,get_param(gcb,'mechspeed'));
      |   polepairs=Simulink.data.evalinGlobal(bdroot,get_param(gcb,'polepairs'));
      |   uscale=Simulink.data.evalinGlobal(bdroot,get_param(gcb,'uscale'));
      |   escale=Simulink.data.evalinGlobal(bdroot,get_param(gcb,'escale'));
      |   iscale=Simulink.data.evalinGlobal(bdroot,get_param(gcb,'iscale'));
      |   if (if0<=0)
      |     warning('Natural frequency f0 must be positive.');
      |   end
      |   if (iksi<=0)
      |     warning('Current loop attenuation must be positive.');
      |   end
      |   if (iksi>1)
      |     warning('Current loop attenuation must not exceed 1.');
      |   end
      |   if (Ld<=0)
      |     warning('Inductance Ld must be positive.');
      |   end
      |   if (Lq<=0)
      |     warning('Inductance Lq must be positive.');
      |   end
      |   if (Rs<0)
      |     warning('Resistance Rs must be non-negative.');
      |   end
      |   if (mechspeed<=0)
      |     warning('Max. speed must be positive.');
      |   end
      |   if (polepairs<1)
      |     warning('Number of pole pairs must be a natural number (1, 2, 3, ...).');
      |   end
      |   if (round(polepairs)~=polepairs)
      |     warning('Number of pole pairs must be a natural number (1, 2, 3, ...).');
      |   end
      |   if (uscale<=0)
      |     warning('U_max must be positive.');
      |   end
      |   if (uscale>escale)
      |     warning('U_max must not exceed E_max');
      |   end
      |   if (iscale<=0)
      |     warning('I_max must be positive.');
      |   end
      |   if (escale<=0)
      |     warning('E_max must be positive.');
      |   end
      |   w0=6.283185307179586*if0;
      |   pgain=2.0*iksi*w0*Ld-Rs;
      |   igain=w0*w0*Ld;
      |   if strcmp(intmethod,'Forward Rectangular')
      |     cc1=pgain;
      |     cc2=-pgain+igain*SampleTime;
      |   else
      |     if strcmp(intmethod,'Backward Rectangular')
      |       cc1=pgain+igain*SampleTime;
      |       cc2=-pgain;
      |     else
      |       cc1=pgain+igain*SampleTime*0.5;
      |       cc2=-pgain+igain*SampleTime*0.5;
      |     end
      |   end
      |   cc1f=cc1*iscale/escale;
      |   cc2f=cc2*iscale/escale;
      |   u16NShift=ceil(log2(abs(cc1f)));
      |   tmpsh=ceil(log2(abs(cc2f)));
      |   if u16NShift<tmpsh
      |     u16NShift=tmpsh;
      |   end
      |   if u16NShift<0
      |     u16NShift=0;
      |   end
      |   if u16NShift>15
      |     u16NShift=15;
      |     warning(['Parameter u16NShift of ' gcb ' exceeds the fixed-point range.']);
      |   end
      |   f16CC1sc_D=round(cc1f*2^(-u16NShift)*2^15);
      |   if f16CC1sc_D>2^15-1
      |     f16CC1sc_D=2^15-1;
      |     warning(['Parameter f16CC1sc_D of ' gcb ' exceeds the fixed-point range.']);
      |   end
      |   if f16CC1sc_D<-2^15
      |     f16CC1sc_D=-2^15;
      |     warning(['Parameter f16CC1sc_D of ' gcb ' exceeds the fixed-point range.']);
      |   end
      |   f16CC2sc_D=round(cc2f*2^(-u16NShift)*2^15);
      |   if f16CC2sc_D>2^15-1
      |     f16CC2sc_D=2^15-1;
      |     warning(['Parameter f16CC2sc_D of ' gcb ' exceeds the fixed-point range.']);
      |   end
      |   if f16CC2sc_D<-2^15
      |     f16CC2sc_D=-2^15;
      |     warning(['Parameter f16CC2sc_D of ' gcb ' exceeds the fixed-point range.']);
      |   end
      |   f16LowerLimit_D=-32768;
      |   f16UpperLimit_D=32767;
      |   f16CC1sc_Q=f16CC1sc_D;
      |   f16CC2sc_Q=f16CC2sc_D;
      |   f16LowerLimit_Q=f16LowerLimit_D;
      |   f16UpperLimit_Q=f16UpperLimit_D;
      |   wmax=polepairs*mechspeed*1.047197551196598e-01;
      |   igainsc=(2.0*Ld-SampleTime*Rs)/(2.0*Ld+SampleTime*Rs);
      |   ugainsc=SampleTime/(2.0*Ld+SampleTime*Rs)*uscale/iscale;
      |   wigainsc=SampleTime*Lq/(2.0*Ld+SampleTime*Rs)*wmax;
      |   egainsc=SampleTime/(2.0*Ld+SampleTime*Rs)*escale/iscale;
      |   maxgain=max(abs([ugainsc,wigainsc,egainsc]));
      |   s16Shift=ceil(log2(abs(maxgain)));
      |   if s16Shift<-15
      |     s16Shift=-15;
      |   end
      |   if s16Shift>15
      |     s16Shift=15;
      |     warning(['Parameter s16Shift of ' gcb ' exceeds the fixed-point range.']);
      |   end
      |   f16IGain=round(igainsc*2^15);
      |   if f16IGain>2^15-1
      |     f16IGain=2^15-1;
      |     warning(['Parameter f16IGain of ' gcb ' exceeds the fixed-point range.']);
      |   end
      |   if f16IGain<-2^15
      |     f16IGain=-2^15;
      |     warning(['Parameter f16IGain of ' gcb ' exceeds the fixed-point range.']);
      |   end
      |   f16UGain=round(ugainsc*2^(-s16Shift)*2^15);
      |   if f16UGain>2^15-1
      |     f16UGain=2^15-1;
      |     warning(['Parameter f16UGain of ' gcb ' exceeds the fixed-point range.']);
      |   end
      |   if f16UGain<-2^15
      |     f16UGain=-2^15;
      |     warning(['Parameter f16UGain of ' gcb ' exceeds the fixed-point range.']);
      |   end
      |   f16WIGain=round(wigainsc*2^(-s16Shift)*2^15);
      |   if f16WIGain>2^15-1
      |     f16WIGain=2^15-1;
      |     warning(['Parameter f16WIGain of ' gcb ' exceeds the fixed-point range.']);
      |   end
      |   if f16WIGain<-2^15
      |     f16WIGain=-2^15;
      |     warning(['Parameter f16WIGain of ' gcb ' exceeds the fixed-point range.']);
      |   end
      |   f16EGain=round(egainsc*2^(-s16Shift)*2^15);
      |   if f16EGain>2^15-1
      |     f16EGain=2^15-1;
      |     warning(['Parameter f16EGain of ' gcb ' exceeds the fixed-point range.']);
      |   end
      |   if f16EGain<-2^15
      |     f16EGain=-2^15;
      |     warning(['Parameter f16EGain of ' gcb ' exceeds the fixed-point range.']);
      |   end
      |   if isnan(f16IGain)
      |     if ~strcmp(f16IGain_bkup,'0')
      |       set_param(gcb,'f16IGain','0');
      |     end
      |   else
      |     tmps=num2str(f16IGain);
      |     if ~strcmp(f16IGain_bkup,tmps)
      |       set_param(gcb,'f16IGain',tmps);
      |     end
      |   end
      |   if isnan(f16UGain)
      |     if ~strcmp(f16UGain_bkup,'0')
      |       set_param(gcb,'f16UGain','0');
      |     end
      |   else
      |     tmps=num2str(f16UGain);
      |     if ~strcmp(f16UGain_bkup,tmps)
      |       set_param(gcb,'f16UGain',tmps);
      |     end
      |   end
      |   if isnan(f16WIGain)
      |     if ~strcmp(f16WIGain_bkup,'0')
      |       set_param(gcb,'f16WIGain','0');
      |     end
      |   else
      |     tmps=num2str(f16WIGain);
      |     if ~strcmp(f16WIGain_bkup,tmps)
      |       set_param(gcb,'f16WIGain',tmps);
      |     end
      |   end
      |   if isnan(f16EGain)
      |     if ~strcmp(f16EGain_bkup,'0')
      |       set_param(gcb,'f16EGain','0');
      |     end
      |   else
      |     tmps=num2str(f16EGain);
      |     if ~strcmp(f16EGain_bkup,tmps)
      |       set_param(gcb,'f16EGain',tmps);
      |     end
      |   end
      |   if isnan(s16Shift)
      |     if ~strcmp(s16Shift_bkup,'0')
      |       set_param(gcb,'s16Shift','0');
      |     end
      |   else
      |     tmps=num2str(s16Shift);
      |     if ~strcmp(s16Shift_bkup,tmps)
      |       set_param(gcb,'s16Shift',tmps);
      |     end
      |   end
      |   if isnan(f16CC1sc_D)
      |     if ~strcmp(f16CC1sc_D_bkup,'0')
      |       set_param(gcb,'f16CC1sc_D','0');
      |     end
      |   else
      |     tmps=num2str(f16CC1sc_D);
      |     if ~strcmp(f16CC1sc_D_bkup,tmps)
      |       set_param(gcb,'f16CC1sc_D',tmps);
      |     end
      |   end
      |   if isnan(f16CC2sc_D)
      |     if ~strcmp(f16CC2sc_D_bkup,'0')
      |       set_param(gcb,'f16CC2sc_D','0');
      |     end
      |   else
      |     tmps=num2str(f16CC2sc_D);
      |     if ~strcmp(f16CC2sc_D_bkup,tmps)
      |       set_param(gcb,'f16CC2sc_D',tmps);
      |     end
      |   end
      |   if isnan(f16UpperLimit_D)
      |     if ~strcmp(f16UpperLimit_D_bkup,'0')
      |       set_param(gcb,'f16UpperLimit_D','0');
      |     end
      |   else
      |     tmps=num2str(f16UpperLimit_D);
      |     if ~strcmp(f16UpperLimit_D_bkup,tmps)
      |       set_param(gcb,'f16UpperLimit_D',tmps);
      |     end
      |   end
      |   if isnan(f16LowerLimit_D)
      |     if ~strcmp(f16LowerLimit_D_bkup,'0')
      |       set_param(gcb,'f16LowerLimit_D','0');
      |     end
      |   else
      |     tmps=num2str(f16LowerLimit_D);
      |     if ~strcmp(f16LowerLimit_D_bkup,tmps)
      |       set_param(gcb,'f16LowerLimit_D',tmps);
      |     end
      |   end
      |   if isnan(f16CC1sc_Q)
      |     if ~strcmp(f16CC1sc_Q_bkup,'0')
      |       set_param(gcb,'f16CC1sc_Q','0');
      |     end
      |   else
      |     tmps=num2str(f16CC1sc_Q);
      |     if ~strcmp(f16CC1sc_Q_bkup,tmps)
      |       set_param(gcb,'f16CC1sc_Q',tmps);
      |     end
      |   end
      |   if isnan(f16CC2sc_Q)
      |     if ~strcmp(f16CC2sc_Q_bkup,'0')
      |       set_param(gcb,'f16CC2sc_Q','0');
      |     end
      |   else
      |     tmps=num2str(f16CC2sc_Q);
      |     if ~strcmp(f16CC2sc_Q_bkup,tmps)
      |       set_param(gcb,'f16CC2sc_Q',tmps);
      |     end
      |   end
      |   if isnan(f16UpperLimit_Q)
      |     if ~strcmp(f16UpperLimit_Q_bkup,'0')
      |       set_param(gcb,'f16UpperLimit_Q','0');
      |     end
      |   else
      |     tmps=num2str(f16UpperLimit_Q);
      |     if ~strcmp(f16UpperLimit_Q_bkup,tmps)
      |       set_param(gcb,'f16UpperLimit_Q',tmps);
      |     end
      |   end
      |   if isnan(f16LowerLimit_Q)
      |     if ~strcmp(f16LowerLimit_Q_bkup,'0')
      |       set_param(gcb,'f16LowerLimit_Q','0');
      |     end
      |   else
      |     tmps=num2str(f16LowerLimit_Q);
      |     if ~strcmp(f16LowerLimit_Q_bkup,tmps)
      |       set_param(gcb,'f16LowerLimit_Q',tmps);
      |     end
      |   end
      |   if isnan(u16NShift)
      |     if ~strcmp(u16NShift_bkup,'0')
      |       set_param(gcb,'u16NShift','0');
      |     end
      |   else
      |     tmps=num2str(u16NShift);
      |     if ~strcmp(u16NShift_bkup,tmps)
      |       set_param(gcb,'u16NShift',tmps);
      |     end
      |   end
      | end
      mask Callback Lq:
      | autoCalcEn=get_param(gcb,'autoCalcEn');
      | if strcmp(autoCalcEn,'on')
      |   SampleTime=Simulink.data.evalinGlobal(bdroot,get_param(gcb,'SampleTime'));
      |   if (SampleTime==-1)
      |     SampleTime=str2double(get_param(gcb,'SampleTime_1'));
      |   end
      |   f16IGain_bkup=get_param(gcb,'f16IGain');
      |   f16UGain_bkup=get_param(gcb,'f16UGain');
      |   f16WIGain_bkup=get_param(gcb,'f16WIGain');
      |   f16EGain_bkup=get_param(gcb,'f16EGain');
      |   s16Shift_bkup=get_param(gcb,'s16Shift');
      |   f16CC1sc_D_bkup=get_param(gcb,'f16CC1sc_D');
      |   f16CC2sc_D_bkup=get_param(gcb,'f16CC2sc_D');
      |   f16UpperLimit_D_bkup=get_param(gcb,'f16UpperLimit_D');
      |   f16LowerLimit_D_bkup=get_param(gcb,'f16LowerLimit_D');
      |   f16CC1sc_Q_bkup=get_param(gcb,'f16CC1sc_Q');
      |   f16CC2sc_Q_bkup=get_param(gcb,'f16CC2sc_Q');
      |   f16UpperLimit_Q_bkup=get_param(gcb,'f16UpperLimit_Q');
      |   f16LowerLimit_Q_bkup=get_param(gcb,'f16LowerLimit_Q');
      |   u16NShift_bkup=get_param(gcb,'u16NShift');
      |   intmethod=get_param(gcb,'intmethod');
      |   if0=Simulink.data.evalinGlobal(bdroot,get_param(gcb,'if0'));
      |   iksi=Simulink.data.evalinGlobal(bdroot,get_param(gcb,'iksi'));
      |   Ld=Simulink.data.evalinGlobal(bdroot,get_param(gcb,'Ld'));
      |   Lq=Simulink.data.evalinGlobal(bdroot,get_param(gcb,'Lq'));
      |   Rs=Simulink.data.evalinGlobal(bdroot,get_param(gcb,'Rs'));
      |   mechspeed=Simulink.data.evalinGlobal(bdroot,get_param(gcb,'mechspeed'));
      |   polepairs=Simulink.data.evalinGlobal(bdroot,get_param(gcb,'polepairs'));
      |   uscale=Simulink.data.evalinGlobal(bdroot,get_param(gcb,'uscale'));
      |   escale=Simulink.data.evalinGlobal(bdroot,get_param(gcb,'escale'));
      |   iscale=Simulink.data.evalinGlobal(bdroot,get_param(gcb,'iscale'));
      |   if (if0<=0)
      |     warning('Natural frequency f0 must be positive.');
      |   end
      |   if (iksi<=0)
      |     warning('Current loop attenuation must be positive.');
      |   end
      |   if (iksi>1)
      |     warning('Current loop attenuation must not exceed 1.');
      |   end
      |   if (Ld<=0)
      |     warning('Inductance Ld must be positive.');
      |   end
      |   if (Lq<=0)
      |     warning('Inductance Lq must be positive.');
      |   end
      |   if (Rs<0)
      |     warning('Resistance Rs must be non-negative.');
      |   end
      |   if (mechspeed<=0)
      |     warning('Max. speed must be positive.');
      |   end
      |   if (polepairs<1)
      |     warning('Number of pole pairs must be a natural number (1, 2, 3, ...).');
      |   end
      |   if (round(polepairs)~=polepairs)
      |     warning('Number of pole pairs must be a natural number (1, 2, 3, ...).');
      |   end
      |   if (uscale<=0)
      |     warning('U_max must be positive.');
      |   end
      |   if (uscale>escale)
      |     warning('U_max must not exceed E_max');
      |   end
      |   if (iscale<=0)
      |     warning('I_max must be positive.');
      |   end
      |   if (escale<=0)
      |     warning('E_max must be positive.');
      |   end
      |   w0=6.283185307179586*if0;
      |   pgain=2.0*iksi*w0*Ld-Rs;
      |   igain=w0*w0*Ld;
      |   if strcmp(intmethod,'Forward Rectangular')
      |     cc1=pgain;
      |     cc2=-pgain+igain*SampleTime;
      |   else
      |     if strcmp(intmethod,'Backward Rectangular')
      |       cc1=pgain+igain*SampleTime;
      |       cc2=-pgain;
      |     else
      |       cc1=pgain+igain*SampleTime*0.5;
      |       cc2=-pgain+igain*SampleTime*0.5;
      |     end
      |   end
      |   cc1f=cc1*iscale/escale;
      |   cc2f=cc2*iscale/escale;
      |   u16NShift=ceil(log2(abs(cc1f)));
      |   tmpsh=ceil(log2(abs(cc2f)));
      |   if u16NShift<tmpsh
      |     u16NShift=tmpsh;
      |   end
      |   if u16NShift<0
      |     u16NShift=0;
      |   end
      |   if u16NShift>15
      |     u16NShift=15;
      |     warning(['Parameter u16NShift of ' gcb ' exceeds the fixed-point range.']);
      |   end
      |   f16CC1sc_D=round(cc1f*2^(-u16NShift)*2^15);
      |   if f16CC1sc_D>2^15-1
      |     f16CC1sc_D=2^15-1;
      |     warning(['Parameter f16CC1sc_D of ' gcb ' exceeds the fixed-point range.']);
      |   end
      |   if f16CC1sc_D<-2^15
      |     f16CC1sc_D=-2^15;
      |     warning(['Parameter f16CC1sc_D of ' gcb ' exceeds the fixed-point range.']);
      |   end
      |   f16CC2sc_D=round(cc2f*2^(-u16NShift)*2^15);
      |   if f16CC2sc_D>2^15-1
      |     f16CC2sc_D=2^15-1;
      |     warning(['Parameter f16CC2sc_D of ' gcb ' exceeds the fixed-point range.']);
      |   end
      |   if f16CC2sc_D<-2^15
      |     f16CC2sc_D=-2^15;
      |     warning(['Parameter f16CC2sc_D of ' gcb ' exceeds the fixed-point range.']);
      |   end
      |   f16LowerLimit_D=-32768;
      |   f16UpperLimit_D=32767;
      |   f16CC1sc_Q=f16CC1sc_D;
      |   f16CC2sc_Q=f16CC2sc_D;
      |   f16LowerLimit_Q=f16LowerLimit_D;
      |   f16UpperLimit_Q=f16UpperLimit_D;
      |   wmax=polepairs*mechspeed*1.047197551196598e-01;
      |   igainsc=(2.0*Ld-SampleTime*Rs)/(2.0*Ld+SampleTime*Rs);
      |   ugainsc=SampleTime/(2.0*Ld+SampleTime*Rs)*uscale/iscale;
      |   wigainsc=SampleTime*Lq/(2.0*Ld+SampleTime*Rs)*wmax;
      |   egainsc=SampleTime/(2.0*Ld+SampleTime*Rs)*escale/iscale;
      |   maxgain=max(abs([ugainsc,wigainsc,egainsc]));
      |   s16Shift=ceil(log2(abs(maxgain)));
      |   if s16Shift<-15
      |     s16Shift=-15;
      |   end
      |   if s16Shift>15
      |     s16Shift=15;
      |     warning(['Parameter s16Shift of ' gcb ' exceeds the fixed-point range.']);
      |   end
      |   f16IGain=round(igainsc*2^15);
      |   if f16IGain>2^15-1
      |     f16IGain=2^15-1;
      |     warning(['Parameter f16IGain of ' gcb ' exceeds the fixed-point range.']);
      |   end
      |   if f16IGain<-2^15
      |     f16IGain=-2^15;
      |     warning(['Parameter f16IGain of ' gcb ' exceeds the fixed-point range.']);
      |   end
      |   f16UGain=round(ugainsc*2^(-s16Shift)*2^15);
      |   if f16UGain>2^15-1
      |     f16UGain=2^15-1;
      |     warning(['Parameter f16UGain of ' gcb ' exceeds the fixed-point range.']);
      |   end
      |   if f16UGain<-2^15
      |     f16UGain=-2^15;
      |     warning(['Parameter f16UGain of ' gcb ' exceeds the fixed-point range.']);
      |   end
      |   f16WIGain=round(wigainsc*2^(-s16Shift)*2^15);
      |   if f16WIGain>2^15-1
      |     f16WIGain=2^15-1;
      |     warning(['Parameter f16WIGain of ' gcb ' exceeds the fixed-point range.']);
      |   end
      |   if f16WIGain<-2^15
      |     f16WIGain=-2^15;
      |     warning(['Parameter f16WIGain of ' gcb ' exceeds the fixed-point range.']);
      |   end
      |   f16EGain=round(egainsc*2^(-s16Shift)*2^15);
      |   if f16EGain>2^15-1
      |     f16EGain=2^15-1;
      |     warning(['Parameter f16EGain of ' gcb ' exceeds the fixed-point range.']);
      |   end
      |   if f16EGain<-2^15
      |     f16EGain=-2^15;
      |     warning(['Parameter f16EGain of ' gcb ' exceeds the fixed-point range.']);
      |   end
      |   if isnan(f16IGain)
      |     if ~strcmp(f16IGain_bkup,'0')
      |       set_param(gcb,'f16IGain','0');
      |     end
      |   else
      |     tmps=num2str(f16IGain);
      |     if ~strcmp(f16IGain_bkup,tmps)
      |       set_param(gcb,'f16IGain',tmps);
      |     end
      |   end
      |   if isnan(f16UGain)
      |     if ~strcmp(f16UGain_bkup,'0')
      |       set_param(gcb,'f16UGain','0');
      |     end
      |   else
      |     tmps=num2str(f16UGain);
      |     if ~strcmp(f16UGain_bkup,tmps)
      |       set_param(gcb,'f16UGain',tmps);
      |     end
      |   end
      |   if isnan(f16WIGain)
      |     if ~strcmp(f16WIGain_bkup,'0')
      |       set_param(gcb,'f16WIGain','0');
      |     end
      |   else
      |     tmps=num2str(f16WIGain);
      |     if ~strcmp(f16WIGain_bkup,tmps)
      |       set_param(gcb,'f16WIGain',tmps);
      |     end
      |   end
      |   if isnan(f16EGain)
      |     if ~strcmp(f16EGain_bkup,'0')
      |       set_param(gcb,'f16EGain','0');
      |     end
      |   else
      |     tmps=num2str(f16EGain);
      |     if ~strcmp(f16EGain_bkup,tmps)
      |       set_param(gcb,'f16EGain',tmps);
      |     end
      |   end
      |   if isnan(s16Shift)
      |     if ~strcmp(s16Shift_bkup,'0')
      |       set_param(gcb,'s16Shift','0');
      |     end
      |   else
      |     tmps=num2str(s16Shift);
      |     if ~strcmp(s16Shift_bkup,tmps)
      |       set_param(gcb,'s16Shift',tmps);
      |     end
      |   end
      |   if isnan(f16CC1sc_D)
      |     if ~strcmp(f16CC1sc_D_bkup,'0')
      |       set_param(gcb,'f16CC1sc_D','0');
      |     end
      |   else
      |     tmps=num2str(f16CC1sc_D);
      |     if ~strcmp(f16CC1sc_D_bkup,tmps)
      |       set_param(gcb,'f16CC1sc_D',tmps);
      |     end
      |   end
      |   if isnan(f16CC2sc_D)
      |     if ~strcmp(f16CC2sc_D_bkup,'0')
      |       set_param(gcb,'f16CC2sc_D','0');
      |     end
      |   else
      |     tmps=num2str(f16CC2sc_D);
      |     if ~strcmp(f16CC2sc_D_bkup,tmps)
      |       set_param(gcb,'f16CC2sc_D',tmps);
      |     end
      |   end
      |   if isnan(f16UpperLimit_D)
      |     if ~strcmp(f16UpperLimit_D_bkup,'0')
      |       set_param(gcb,'f16UpperLimit_D','0');
      |     end
      |   else
      |     tmps=num2str(f16UpperLimit_D);
      |     if ~strcmp(f16UpperLimit_D_bkup,tmps)
      |       set_param(gcb,'f16UpperLimit_D',tmps);
      |     end
      |   end
      |   if isnan(f16LowerLimit_D)
      |     if ~strcmp(f16LowerLimit_D_bkup,'0')
      |       set_param(gcb,'f16LowerLimit_D','0');
      |     end
      |   else
      |     tmps=num2str(f16LowerLimit_D);
      |     if ~strcmp(f16LowerLimit_D_bkup,tmps)
      |       set_param(gcb,'f16LowerLimit_D',tmps);
      |     end
      |   end
      |   if isnan(f16CC1sc_Q)
      |     if ~strcmp(f16CC1sc_Q_bkup,'0')
      |       set_param(gcb,'f16CC1sc_Q','0');
      |     end
      |   else
      |     tmps=num2str(f16CC1sc_Q);
      |     if ~strcmp(f16CC1sc_Q_bkup,tmps)
      |       set_param(gcb,'f16CC1sc_Q',tmps);
      |     end
      |   end
      |   if isnan(f16CC2sc_Q)
      |     if ~strcmp(f16CC2sc_Q_bkup,'0')
      |       set_param(gcb,'f16CC2sc_Q','0');
      |     end
      |   else
      |     tmps=num2str(f16CC2sc_Q);
      |     if ~strcmp(f16CC2sc_Q_bkup,tmps)
      |       set_param(gcb,'f16CC2sc_Q',tmps);
      |     end
      |   end
      |   if isnan(f16UpperLimit_Q)
      |     if ~strcmp(f16UpperLimit_Q_bkup,'0')
      |       set_param(gcb,'f16UpperLimit_Q','0');
      |     end
      |   else
      |     tmps=num2str(f16UpperLimit_Q);
      |     if ~strcmp(f16UpperLimit_Q_bkup,tmps)
      |       set_param(gcb,'f16UpperLimit_Q',tmps);
      |     end
      |   end
      |   if isnan(f16LowerLimit_Q)
      |     if ~strcmp(f16LowerLimit_Q_bkup,'0')
      |       set_param(gcb,'f16LowerLimit_Q','0');
      |     end
      |   else
      |     tmps=num2str(f16LowerLimit_Q);
      |     if ~strcmp(f16LowerLimit_Q_bkup,tmps)
      |       set_param(gcb,'f16LowerLimit_Q',tmps);
      |     end
      |   end
      |   if isnan(u16NShift)
      |     if ~strcmp(u16NShift_bkup,'0')
      |       set_param(gcb,'u16NShift','0');
      |     end
      |   else
      |     tmps=num2str(u16NShift);
      |     if ~strcmp(u16NShift_bkup,tmps)
      |       set_param(gcb,'u16NShift',tmps);
      |     end
      |   end
      | end
      mask Callback Rs:
      | autoCalcEn=get_param(gcb,'autoCalcEn');
      | if strcmp(autoCalcEn,'on')
      |   SampleTime=Simulink.data.evalinGlobal(bdroot,get_param(gcb,'SampleTime'));
      |   if (SampleTime==-1)
      |     SampleTime=str2double(get_param(gcb,'SampleTime_1'));
      |   end
      |   f16IGain_bkup=get_param(gcb,'f16IGain');
      |   f16UGain_bkup=get_param(gcb,'f16UGain');
      |   f16WIGain_bkup=get_param(gcb,'f16WIGain');
      |   f16EGain_bkup=get_param(gcb,'f16EGain');
      |   s16Shift_bkup=get_param(gcb,'s16Shift');
      |   f16CC1sc_D_bkup=get_param(gcb,'f16CC1sc_D');
      |   f16CC2sc_D_bkup=get_param(gcb,'f16CC2sc_D');
      |   f16UpperLimit_D_bkup=get_param(gcb,'f16UpperLimit_D');
      |   f16LowerLimit_D_bkup=get_param(gcb,'f16LowerLimit_D');
      |   f16CC1sc_Q_bkup=get_param(gcb,'f16CC1sc_Q');
      |   f16CC2sc_Q_bkup=get_param(gcb,'f16CC2sc_Q');
      |   f16UpperLimit_Q_bkup=get_param(gcb,'f16UpperLimit_Q');
      |   f16LowerLimit_Q_bkup=get_param(gcb,'f16LowerLimit_Q');
      |   u16NShift_bkup=get_param(gcb,'u16NShift');
      |   intmethod=get_param(gcb,'intmethod');
      |   if0=Simulink.data.evalinGlobal(bdroot,get_param(gcb,'if0'));
      |   iksi=Simulink.data.evalinGlobal(bdroot,get_param(gcb,'iksi'));
      |   Ld=Simulink.data.evalinGlobal(bdroot,get_param(gcb,'Ld'));
      |   Lq=Simulink.data.evalinGlobal(bdroot,get_param(gcb,'Lq'));
      |   Rs=Simulink.data.evalinGlobal(bdroot,get_param(gcb,'Rs'));
      |   mechspeed=Simulink.data.evalinGlobal(bdroot,get_param(gcb,'mechspeed'));
      |   polepairs=Simulink.data.evalinGlobal(bdroot,get_param(gcb,'polepairs'));
      |   uscale=Simulink.data.evalinGlobal(bdroot,get_param(gcb,'uscale'));
      |   escale=Simulink.data.evalinGlobal(bdroot,get_param(gcb,'escale'));
      |   iscale=Simulink.data.evalinGlobal(bdroot,get_param(gcb,'iscale'));
      |   if (if0<=0)
      |     warning('Natural frequency f0 must be positive.');
      |   end
      |   if (iksi<=0)
      |     warning('Current loop attenuation must be positive.');
      |   end
      |   if (iksi>1)
      |     warning('Current loop attenuation must not exceed 1.');
      |   end
      |   if (Ld<=0)
      |     warning('Inductance Ld must be positive.');
      |   end
      |   if (Lq<=0)
      |     warning('Inductance Lq must be positive.');
      |   end
      |   if (Rs<0)
      |     warning('Resistance Rs must be non-negative.');
      |   end
      |   if (mechspeed<=0)
      |     warning('Max. speed must be positive.');
      |   end
      |   if (polepairs<1)
      |     warning('Number of pole pairs must be a natural number (1, 2, 3, ...).');
      |   end
      |   if (round(polepairs)~=polepairs)
      |     warning('Number of pole pairs must be a natural number (1, 2, 3, ...).');
      |   end
      |   if (uscale<=0)
      |     warning('U_max must be positive.');
      |   end
      |   if (uscale>escale)
      |     warning('U_max must not exceed E_max');
      |   end
      |   if (iscale<=0)
      |     warning('I_max must be positive.');
      |   end
      |   if (escale<=0)
      |     warning('E_max must be positive.');
      |   end
      |   w0=6.283185307179586*if0;
      |   pgain=2.0*iksi*w0*Ld-Rs;
      |   igain=w0*w0*Ld;
      |   if strcmp(intmethod,'Forward Rectangular')
      |     cc1=pgain;
      |     cc2=-pgain+igain*SampleTime;
      |   else
      |     if strcmp(intmethod,'Backward Rectangular')
      |       cc1=pgain+igain*SampleTime;
      |       cc2=-pgain;
      |     else
      |       cc1=pgain+igain*SampleTime*0.5;
      |       cc2=-pgain+igain*SampleTime*0.5;
      |     end
      |   end
      |   cc1f=cc1*iscale/escale;
      |   cc2f=cc2*iscale/escale;
      |   u16NShift=ceil(log2(abs(cc1f)));
      |   tmpsh=ceil(log2(abs(cc2f)));
      |   if u16NShift<tmpsh
      |     u16NShift=tmpsh;
      |   end
      |   if u16NShift<0
      |     u16NShift=0;
      |   end
      |   if u16NShift>15
      |     u16NShift=15;
      |     warning(['Parameter u16NShift of ' gcb ' exceeds the fixed-point range.']);
      |   end
      |   f16CC1sc_D=round(cc1f*2^(-u16NShift)*2^15);
      |   if f16CC1sc_D>2^15-1
      |     f16CC1sc_D=2^15-1;
      |     warning(['Parameter f16CC1sc_D of ' gcb ' exceeds the fixed-point range.']);
      |   end
      |   if f16CC1sc_D<-2^15
      |     f16CC1sc_D=-2^15;
      |     warning(['Parameter f16CC1sc_D of ' gcb ' exceeds the fixed-point range.']);
      |   end
      |   f16CC2sc_D=round(cc2f*2^(-u16NShift)*2^15);
      |   if f16CC2sc_D>2^15-1
      |     f16CC2sc_D=2^15-1;
      |     warning(['Parameter f16CC2sc_D of ' gcb ' exceeds the fixed-point range.']);
      |   end
      |   if f16CC2sc_D<-2^15
      |     f16CC2sc_D=-2^15;
      |     warning(['Parameter f16CC2sc_D of ' gcb ' exceeds the fixed-point range.']);
      |   end
      |   f16LowerLimit_D=-32768;
      |   f16UpperLimit_D=32767;
      |   f16CC1sc_Q=f16CC1sc_D;
      |   f16CC2sc_Q=f16CC2sc_D;
      |   f16LowerLimit_Q=f16LowerLimit_D;
      |   f16UpperLimit_Q=f16UpperLimit_D;
      |   wmax=polepairs*mechspeed*1.047197551196598e-01;
      |   igainsc=(2.0*Ld-SampleTime*Rs)/(2.0*Ld+SampleTime*Rs);
      |   ugainsc=SampleTime/(2.0*Ld+SampleTime*Rs)*uscale/iscale;
      |   wigainsc=SampleTime*Lq/(2.0*Ld+SampleTime*Rs)*wmax;
      |   egainsc=SampleTime/(2.0*Ld+SampleTime*Rs)*escale/iscale;
      |   maxgain=max(abs([ugainsc,wigainsc,egainsc]));
      |   s16Shift=ceil(log2(abs(maxgain)));
      |   if s16Shift<-15
      |     s16Shift=-15;
      |   end
      |   if s16Shift>15
      |     s16Shift=15;
      |     warning(['Parameter s16Shift of ' gcb ' exceeds the fixed-point range.']);
      |   end
      |   f16IGain=round(igainsc*2^15);
      |   if f16IGain>2^15-1
      |     f16IGain=2^15-1;
      |     warning(['Parameter f16IGain of ' gcb ' exceeds the fixed-point range.']);
      |   end
      |   if f16IGain<-2^15
      |     f16IGain=-2^15;
      |     warning(['Parameter f16IGain of ' gcb ' exceeds the fixed-point range.']);
      |   end
      |   f16UGain=round(ugainsc*2^(-s16Shift)*2^15);
      |   if f16UGain>2^15-1
      |     f16UGain=2^15-1;
      |     warning(['Parameter f16UGain of ' gcb ' exceeds the fixed-point range.']);
      |   end
      |   if f16UGain<-2^15
      |     f16UGain=-2^15;
      |     warning(['Parameter f16UGain of ' gcb ' exceeds the fixed-point range.']);
      |   end
      |   f16WIGain=round(wigainsc*2^(-s16Shift)*2^15);
      |   if f16WIGain>2^15-1
      |     f16WIGain=2^15-1;
      |     warning(['Parameter f16WIGain of ' gcb ' exceeds the fixed-point range.']);
      |   end
      |   if f16WIGain<-2^15
      |     f16WIGain=-2^15;
      |     warning(['Parameter f16WIGain of ' gcb ' exceeds the fixed-point range.']);
      |   end
      |   f16EGain=round(egainsc*2^(-s16Shift)*2^15);
      |   if f16EGain>2^15-1
      |     f16EGain=2^15-1;
      |     warning(['Parameter f16EGain of ' gcb ' exceeds the fixed-point range.']);
      |   end
      |   if f16EGain<-2^15
      |     f16EGain=-2^15;
      |     warning(['Parameter f16EGain of ' gcb ' exceeds the fixed-point range.']);
      |   end
      |   if isnan(f16IGain)
      |     if ~strcmp(f16IGain_bkup,'0')
      |       set_param(gcb,'f16IGain','0');
      |     end
      |   else
      |     tmps=num2str(f16IGain);
      |     if ~strcmp(f16IGain_bkup,tmps)
      |       set_param(gcb,'f16IGain',tmps);
      |     end
      |   end
      |   if isnan(f16UGain)
      |     if ~strcmp(f16UGain_bkup,'0')
      |       set_param(gcb,'f16UGain','0');
      |     end
      |   else
      |     tmps=num2str(f16UGain);
      |     if ~strcmp(f16UGain_bkup,tmps)
      |       set_param(gcb,'f16UGain',tmps);
      |     end
      |   end
      |   if isnan(f16WIGain)
      |     if ~strcmp(f16WIGain_bkup,'0')
      |       set_param(gcb,'f16WIGain','0');
      |     end
      |   else
      |     tmps=num2str(f16WIGain);
      |     if ~strcmp(f16WIGain_bkup,tmps)
      |       set_param(gcb,'f16WIGain',tmps);
      |     end
      |   end
      |   if isnan(f16EGain)
      |     if ~strcmp(f16EGain_bkup,'0')
      |       set_param(gcb,'f16EGain','0');
      |     end
      |   else
      |     tmps=num2str(f16EGain);
      |     if ~strcmp(f16EGain_bkup,tmps)
      |       set_param(gcb,'f16EGain',tmps);
      |     end
      |   end
      |   if isnan(s16Shift)
      |     if ~strcmp(s16Shift_bkup,'0')
      |       set_param(gcb,'s16Shift','0');
      |     end
      |   else
      |     tmps=num2str(s16Shift);
      |     if ~strcmp(s16Shift_bkup,tmps)
      |       set_param(gcb,'s16Shift',tmps);
      |     end
      |   end
      |   if isnan(f16CC1sc_D)
      |     if ~strcmp(f16CC1sc_D_bkup,'0')
      |       set_param(gcb,'f16CC1sc_D','0');
      |     end
      |   else
      |     tmps=num2str(f16CC1sc_D);
      |     if ~strcmp(f16CC1sc_D_bkup,tmps)
      |       set_param(gcb,'f16CC1sc_D',tmps);
      |     end
      |   end
      |   if isnan(f16CC2sc_D)
      |     if ~strcmp(f16CC2sc_D_bkup,'0')
      |       set_param(gcb,'f16CC2sc_D','0');
      |     end
      |   else
      |     tmps=num2str(f16CC2sc_D);
      |     if ~strcmp(f16CC2sc_D_bkup,tmps)
      |       set_param(gcb,'f16CC2sc_D',tmps);
      |     end
      |   end
      |   if isnan(f16UpperLimit_D)
      |     if ~strcmp(f16UpperLimit_D_bkup,'0')
      |       set_param(gcb,'f16UpperLimit_D','0');
      |     end
      |   else
      |     tmps=num2str(f16UpperLimit_D);
      |     if ~strcmp(f16UpperLimit_D_bkup,tmps)
      |       set_param(gcb,'f16UpperLimit_D',tmps);
      |     end
      |   end
      |   if isnan(f16LowerLimit_D)
      |     if ~strcmp(f16LowerLimit_D_bkup,'0')
      |       set_param(gcb,'f16LowerLimit_D','0');
      |     end
      |   else
      |     tmps=num2str(f16LowerLimit_D);
      |     if ~strcmp(f16LowerLimit_D_bkup,tmps)
      |       set_param(gcb,'f16LowerLimit_D',tmps);
      |     end
      |   end
      |   if isnan(f16CC1sc_Q)
      |     if ~strcmp(f16CC1sc_Q_bkup,'0')
      |       set_param(gcb,'f16CC1sc_Q','0');
      |     end
      |   else
      |     tmps=num2str(f16CC1sc_Q);
      |     if ~strcmp(f16CC1sc_Q_bkup,tmps)
      |       set_param(gcb,'f16CC1sc_Q',tmps);
      |     end
      |   end
      |   if isnan(f16CC2sc_Q)
      |     if ~strcmp(f16CC2sc_Q_bkup,'0')
      |       set_param(gcb,'f16CC2sc_Q','0');
      |     end
      |   else
      |     tmps=num2str(f16CC2sc_Q);
      |     if ~strcmp(f16CC2sc_Q_bkup,tmps)
      |       set_param(gcb,'f16CC2sc_Q',tmps);
      |     end
      |   end
      |   if isnan(f16UpperLimit_Q)
      |     if ~strcmp(f16UpperLimit_Q_bkup,'0')
      |       set_param(gcb,'f16UpperLimit_Q','0');
      |     end
      |   else
      |     tmps=num2str(f16UpperLimit_Q);
      |     if ~strcmp(f16UpperLimit_Q_bkup,tmps)
      |       set_param(gcb,'f16UpperLimit_Q',tmps);
      |     end
      |   end
      |   if isnan(f16LowerLimit_Q)
      |     if ~strcmp(f16LowerLimit_Q_bkup,'0')
      |       set_param(gcb,'f16LowerLimit_Q','0');
      |     end
      |   else
      |     tmps=num2str(f16LowerLimit_Q);
      |     if ~strcmp(f16LowerLimit_Q_bkup,tmps)
      |       set_param(gcb,'f16LowerLimit_Q',tmps);
      |     end
      |   end
      |   if isnan(u16NShift)
      |     if ~strcmp(u16NShift_bkup,'0')
      |       set_param(gcb,'u16NShift','0');
      |     end
      |   else
      |     tmps=num2str(u16NShift);
      |     if ~strcmp(u16NShift_bkup,tmps)
      |       set_param(gcb,'u16NShift',tmps);
      |     end
      |   end
      | end
      mask Callback mechspeed:
      | autoCalcEn=get_param(gcb,'autoCalcEn');
      | if strcmp(autoCalcEn,'on')
      |   SampleTime=Simulink.data.evalinGlobal(bdroot,get_param(gcb,'SampleTime'));
      |   if (SampleTime==-1)
      |     SampleTime=str2double(get_param(gcb,'SampleTime_1'));
      |   end
      |   f16IGain_bkup=get_param(gcb,'f16IGain');
      |   f16UGain_bkup=get_param(gcb,'f16UGain');
      |   f16WIGain_bkup=get_param(gcb,'f16WIGain');
      |   f16EGain_bkup=get_param(gcb,'f16EGain');
      |   s16Shift_bkup=get_param(gcb,'s16Shift');
      |   f16CC1sc_D_bkup=get_param(gcb,'f16CC1sc_D');
      |   f16CC2sc_D_bkup=get_param(gcb,'f16CC2sc_D');
      |   f16UpperLimit_D_bkup=get_param(gcb,'f16UpperLimit_D');
      |   f16LowerLimit_D_bkup=get_param(gcb,'f16LowerLimit_D');
      |   f16CC1sc_Q_bkup=get_param(gcb,'f16CC1sc_Q');
      |   f16CC2sc_Q_bkup=get_param(gcb,'f16CC2sc_Q');
      |   f16UpperLimit_Q_bkup=get_param(gcb,'f16UpperLimit_Q');
      |   f16LowerLimit_Q_bkup=get_param(gcb,'f16LowerLimit_Q');
      |   u16NShift_bkup=get_param(gcb,'u16NShift');
      |   intmethod=get_param(gcb,'intmethod');
      |   if0=Simulink.data.evalinGlobal(bdroot,get_param(gcb,'if0'));
      |   iksi=Simulink.data.evalinGlobal(bdroot,get_param(gcb,'iksi'));
      |   Ld=Simulink.data.evalinGlobal(bdroot,get_param(gcb,'Ld'));
      |   Lq=Simulink.data.evalinGlobal(bdroot,get_param(gcb,'Lq'));
      |   Rs=Simulink.data.evalinGlobal(bdroot,get_param(gcb,'Rs'));
      |   mechspeed=Simulink.data.evalinGlobal(bdroot,get_param(gcb,'mechspeed'));
      |   polepairs=Simulink.data.evalinGlobal(bdroot,get_param(gcb,'polepairs'));
      |   uscale=Simulink.data.evalinGlobal(bdroot,get_param(gcb,'uscale'));
      |   escale=Simulink.data.evalinGlobal(bdroot,get_param(gcb,'escale'));
      |   iscale=Simulink.data.evalinGlobal(bdroot,get_param(gcb,'iscale'));
      |   if (if0<=0)
      |     warning('Natural frequency f0 must be positive.');
      |   end
      |   if (iksi<=0)
      |     warning('Current loop attenuation must be positive.');
      |   end
      |   if (iksi>1)
      |     warning('Current loop attenuation must not exceed 1.');
      |   end
      |   if (Ld<=0)
      |     warning('Inductance Ld must be positive.');
      |   end
      |   if (Lq<=0)
      |     warning('Inductance Lq must be positive.');
      |   end
      |   if (Rs<0)
      |     warning('Resistance Rs must be non-negative.');
      |   end
      |   if (mechspeed<=0)
      |     warning('Max. speed must be positive.');
      |   end
      |   if (polepairs<1)
      |     warning('Number of pole pairs must be a natural number (1, 2, 3, ...).');
      |   end
      |   if (round(polepairs)~=polepairs)
      |     warning('Number of pole pairs must be a natural number (1, 2, 3, ...).');
      |   end
      |   if (uscale<=0)
      |     warning('U_max must be positive.');
      |   end
      |   if (uscale>escale)
      |     warning('U_max must not exceed E_max');
      |   end
      |   if (iscale<=0)
      |     warning('I_max must be positive.');
      |   end
      |   if (escale<=0)
      |     warning('E_max must be positive.');
      |   end
      |   w0=6.283185307179586*if0;
      |   pgain=2.0*iksi*w0*Ld-Rs;
      |   igain=w0*w0*Ld;
      |   if strcmp(intmethod,'Forward Rectangular')
      |     cc1=pgain;
      |     cc2=-pgain+igain*SampleTime;
      |   else
      |     if strcmp(intmethod,'Backward Rectangular')
      |       cc1=pgain+igain*SampleTime;
      |       cc2=-pgain;
      |     else
      |       cc1=pgain+igain*SampleTime*0.5;
      |       cc2=-pgain+igain*SampleTime*0.5;
      |     end
      |   end
      |   cc1f=cc1*iscale/escale;
      |   cc2f=cc2*iscale/escale;
      |   u16NShift=ceil(log2(abs(cc1f)));
      |   tmpsh=ceil(log2(abs(cc2f)));
      |   if u16NShift<tmpsh
      |     u16NShift=tmpsh;
      |   end
      |   if u16NShift<0
      |     u16NShift=0;
      |   end
      |   if u16NShift>15
      |     u16NShift=15;
      |     warning(['Parameter u16NShift of ' gcb ' exceeds the fixed-point range.']);
      |   end
      |   f16CC1sc_D=round(cc1f*2^(-u16NShift)*2^15);
      |   if f16CC1sc_D>2^15-1
      |     f16CC1sc_D=2^15-1;
      |     warning(['Parameter f16CC1sc_D of ' gcb ' exceeds the fixed-point range.']);
      |   end
      |   if f16CC1sc_D<-2^15
      |     f16CC1sc_D=-2^15;
      |     warning(['Parameter f16CC1sc_D of ' gcb ' exceeds the fixed-point range.']);
      |   end
      |   f16CC2sc_D=round(cc2f*2^(-u16NShift)*2^15);
      |   if f16CC2sc_D>2^15-1
      |     f16CC2sc_D=2^15-1;
      |     warning(['Parameter f16CC2sc_D of ' gcb ' exceeds the fixed-point range.']);
      |   end
      |   if f16CC2sc_D<-2^15
      |     f16CC2sc_D=-2^15;
      |     warning(['Parameter f16CC2sc_D of ' gcb ' exceeds the fixed-point range.']);
      |   end
      |   f16LowerLimit_D=-32768;
      |   f16UpperLimit_D=32767;
      |   f16CC1sc_Q=f16CC1sc_D;
      |   f16CC2sc_Q=f16CC2sc_D;
      |   f16LowerLimit_Q=f16LowerLimit_D;
      |   f16UpperLimit_Q=f16UpperLimit_D;
      |   wmax=polepairs*mechspeed*1.047197551196598e-01;
      |   igainsc=(2.0*Ld-SampleTime*Rs)/(2.0*Ld+SampleTime*Rs);
      |   ugainsc=SampleTime/(2.0*Ld+SampleTime*Rs)*uscale/iscale;
      |   wigainsc=SampleTime*Lq/(2.0*Ld+SampleTime*Rs)*wmax;
      |   egainsc=SampleTime/(2.0*Ld+SampleTime*Rs)*escale/iscale;
      |   maxgain=max(abs([ugainsc,wigainsc,egainsc]));
      |   s16Shift=ceil(log2(abs(maxgain)));
      |   if s16Shift<-15
      |     s16Shift=-15;
      |   end
      |   if s16Shift>15
      |     s16Shift=15;
      |     warning(['Parameter s16Shift of ' gcb ' exceeds the fixed-point range.']);
      |   end
      |   f16IGain=round(igainsc*2^15);
      |   if f16IGain>2^15-1
      |     f16IGain=2^15-1;
      |     warning(['Parameter f16IGain of ' gcb ' exceeds the fixed-point range.']);
      |   end
      |   if f16IGain<-2^15
      |     f16IGain=-2^15;
      |     warning(['Parameter f16IGain of ' gcb ' exceeds the fixed-point range.']);
      |   end
      |   f16UGain=round(ugainsc*2^(-s16Shift)*2^15);
      |   if f16UGain>2^15-1
      |     f16UGain=2^15-1;
      |     warning(['Parameter f16UGain of ' gcb ' exceeds the fixed-point range.']);
      |   end
      |   if f16UGain<-2^15
      |     f16UGain=-2^15;
      |     warning(['Parameter f16UGain of ' gcb ' exceeds the fixed-point range.']);
      |   end
      |   f16WIGain=round(wigainsc*2^(-s16Shift)*2^15);
      |   if f16WIGain>2^15-1
      |     f16WIGain=2^15-1;
      |     warning(['Parameter f16WIGain of ' gcb ' exceeds the fixed-point range.']);
      |   end
      |   if f16WIGain<-2^15
      |     f16WIGain=-2^15;
      |     warning(['Parameter f16WIGain of ' gcb ' exceeds the fixed-point range.']);
      |   end
      |   f16EGain=round(egainsc*2^(-s16Shift)*2^15);
      |   if f16EGain>2^15-1
      |     f16EGain=2^15-1;
      |     warning(['Parameter f16EGain of ' gcb ' exceeds the fixed-point range.']);
      |   end
      |   if f16EGain<-2^15
      |     f16EGain=-2^15;
      |     warning(['Parameter f16EGain of ' gcb ' exceeds the fixed-point range.']);
      |   end
      |   if isnan(f16IGain)
      |     if ~strcmp(f16IGain_bkup,'0')
      |       set_param(gcb,'f16IGain','0');
      |     end
      |   else
      |     tmps=num2str(f16IGain);
      |     if ~strcmp(f16IGain_bkup,tmps)
      |       set_param(gcb,'f16IGain',tmps);
      |     end
      |   end
      |   if isnan(f16UGain)
      |     if ~strcmp(f16UGain_bkup,'0')
      |       set_param(gcb,'f16UGain','0');
      |     end
      |   else
      |     tmps=num2str(f16UGain);
      |     if ~strcmp(f16UGain_bkup,tmps)
      |       set_param(gcb,'f16UGain',tmps);
      |     end
      |   end
      |   if isnan(f16WIGain)
      |     if ~strcmp(f16WIGain_bkup,'0')
      |       set_param(gcb,'f16WIGain','0');
      |     end
      |   else
      |     tmps=num2str(f16WIGain);
      |     if ~strcmp(f16WIGain_bkup,tmps)
      |       set_param(gcb,'f16WIGain',tmps);
      |     end
      |   end
      |   if isnan(f16EGain)
      |     if ~strcmp(f16EGain_bkup,'0')
      |       set_param(gcb,'f16EGain','0');
      |     end
      |   else
      |     tmps=num2str(f16EGain);
      |     if ~strcmp(f16EGain_bkup,tmps)
      |       set_param(gcb,'f16EGain',tmps);
      |     end
      |   end
      |   if isnan(s16Shift)
      |     if ~strcmp(s16Shift_bkup,'0')
      |       set_param(gcb,'s16Shift','0');
      |     end
      |   else
      |     tmps=num2str(s16Shift);
      |     if ~strcmp(s16Shift_bkup,tmps)
      |       set_param(gcb,'s16Shift',tmps);
      |     end
      |   end
      |   if isnan(f16CC1sc_D)
      |     if ~strcmp(f16CC1sc_D_bkup,'0')
      |       set_param(gcb,'f16CC1sc_D','0');
      |     end
      |   else
      |     tmps=num2str(f16CC1sc_D);
      |     if ~strcmp(f16CC1sc_D_bkup,tmps)
